simulink library "ammclib_bam_S32K3xx"  (R2016a)
(part 5 of 50)

      |     u16NShift_Q=15;
      |     warning(['Parameter u16NShift_Q of ' gcb ' exceeds the fixed-point range.']);
      |   end
      |   f16CC1sc_D=round(cc1fd*2^(-u16NShift_D)*2^15);
      |   if f16CC1sc_D>2^15-1
      |     f16CC1sc_D=2^15-1;
      |     warning(['Parameter f16CC1sc_D of ' gcb ' exceeds the fixed-point range.']);
      |   end
      |   if f16CC1sc_D<-2^15
      |     f16CC1sc_D=-2^15;
      |     warning(['Parameter f16CC1sc_D of ' gcb ' exceeds the fixed-point range.']);
      |   end
      |   f16CC2sc_D=round(cc2fd*2^(-u16NShift_D)*2^15);
      |   if f16CC2sc_D>2^15-1
      |     f16CC2sc_D=2^15-1;
      |     warning(['Parameter f16CC2sc_D of ' gcb ' exceeds the fixed-point range.']);
      |   end
      |   if f16CC2sc_D<-2^15
      |     f16CC2sc_D=-2^15;
      |     warning(['Parameter f16CC2sc_D of ' gcb ' exceeds the fixed-point range.']);
      |   end
      |   f16CC1sc_Q=round(cc1fq*2^(-u16NShift_Q)*2^15);
      |   if f16CC1sc_Q>2^15-1
      |     f16CC1sc_Q=2^15-1;
      |     warning(['Parameter f16CC1sc_Q of ' gcb ' exceeds the fixed-point range.']);
      |   end
      |   if f16CC1sc_Q<-2^15
      |     f16CC1sc_Q=-2^15;
      |     warning(['Parameter f16CC1sc_Q of ' gcb ' exceeds the fixed-point range.']);
      |   end
      |   f16CC2sc_Q=round(cc2fq*2^(-u16NShift_Q)*2^15);
      |   if f16CC2sc_Q>2^15-1
      |     f16CC2sc_Q=2^15-1;
      |     warning(['Parameter f16CC2sc_Q of ' gcb ' exceeds the fixed-point range.']);
      |   end
      |   if f16CC2sc_Q<-2^15
      |     f16CC2sc_Q=-2^15;
      |     warning(['Parameter f16CC2sc_Q of ' gcb ' exceeds the fixed-point range.']);
      |   end
      |   if isnan(f16CC1sc_D)
      |     if ~strcmp(f16CC1sc_D_bkup,'0')
      |       set_param(gcb,'f16CC1sc_D','0');
      |     end
      |   else
      |     tmps=num2str(f16CC1sc_D);
      |     if ~strcmp(f16CC1sc_D_bkup,tmps)
      |       set_param(gcb,'f16CC1sc_D',tmps);
      |     end
      |   end
      |   if isnan(f16CC2sc_D)
      |     if ~strcmp(f16CC2sc_D_bkup,'0')
      |       set_param(gcb,'f16CC2sc_D','0');
      |     end
      |   else
      |     tmps=num2str(f16CC2sc_D);
      |     if ~strcmp(f16CC2sc_D_bkup,tmps)
      |       set_param(gcb,'f16CC2sc_D',tmps);
      |     end
      |   end
      |   if isnan(u16NShift_D)
      |     if ~strcmp(u16NShift_D_bkup,'0')
      |       set_param(gcb,'u16NShift_D','0');
      |     end
      |   else
      |     tmps=num2str(u16NShift_D);
      |     if ~strcmp(u16NShift_D_bkup,tmps)
      |       set_param(gcb,'u16NShift_D',tmps);
      |     end
      |   end
      |   if isnan(f16CC1sc_Q)
      |     if ~strcmp(f16CC1sc_Q_bkup,'0')
      |       set_param(gcb,'f16CC1sc_Q','0');
      |     end
      |   else
      |     tmps=num2str(f16CC1sc_Q);
      |     if ~strcmp(f16CC1sc_Q_bkup,tmps)
      |       set_param(gcb,'f16CC1sc_Q',tmps);
      |     end
      |   end
      |   if isnan(f16CC2sc_Q)
      |     if ~strcmp(f16CC2sc_Q_bkup,'0')
      |       set_param(gcb,'f16CC2sc_Q','0');
      |     end
      |   else
      |     tmps=num2str(f16CC2sc_Q);
      |     if ~strcmp(f16CC2sc_Q_bkup,tmps)
      |       set_param(gcb,'f16CC2sc_Q',tmps);
      |     end
      |   end
      |   if isnan(u16NShift_Q)
      |     if ~strcmp(u16NShift_Q_bkup,'0')
      |       set_param(gcb,'u16NShift_Q','0');
      |     end
      |   else
      |     tmps=num2str(u16NShift_Q);
      |     if ~strcmp(u16NShift_Q_bkup,tmps)
      |       set_param(gcb,'u16NShift_Q',tmps);
      |     end
      |   end
      | end
      mask Callback iscale:
      | autoCalcEn=get_param(gcb,'autoCalcEn');
      | if strcmp(autoCalcEn,'on')
      |   SampleTime=Simulink.data.evalinGlobal(bdroot,get_param(gcb,'SampleTime'));
      |   if (SampleTime==-1)
      |     SampleTime=str2double(get_param(gcb,'SampleTime_1'));
      |   end
      |   f16CC1sc_D_bkup=get_param(gcb,'f16CC1sc_D');
      |   f16CC2sc_D_bkup=get_param(gcb,'f16CC2sc_D');
      |   u16NShift_D_bkup=get_param(gcb,'u16NShift_D');
      |   f16CC1sc_Q_bkup=get_param(gcb,'f16CC1sc_Q');
      |   f16CC2sc_Q_bkup=get_param(gcb,'f16CC2sc_Q');
      |   u16NShift_Q_bkup=get_param(gcb,'u16NShift_Q');
      |   intmethod=get_param(gcb,'intmethod');
      |   if0=Simulink.data.evalinGlobal(bdroot,get_param(gcb,'if0'));
      |   iksi=Simulink.data.evalinGlobal(bdroot,get_param(gcb,'iksi'));
      |   Ld=Simulink.data.evalinGlobal(bdroot,get_param(gcb,'Ld'));
      |   Lq=Simulink.data.evalinGlobal(bdroot,get_param(gcb,'Lq'));
      |   Rs=Simulink.data.evalinGlobal(bdroot,get_param(gcb,'Rs'));
      |   uscale=Simulink.data.evalinGlobal(bdroot,get_param(gcb,'uscale'));
      |   iscale=Simulink.data.evalinGlobal(bdroot,get_param(gcb,'iscale'));
      |   if (if0<=0)
      |     warning('Natural frequency f0 must be positive.');
      |   end
      |   if (iksi<=0)
      |     warning('Current loop attenuation must be positive.');
      |   end
      |   if (iksi>1)
      |     warning('Current loop attenuation must not exceed 1.');
      |   end
      |   if (Ld<=0)
      |     warning('Inductance Ld must be positive.');
      |   end
      |   if (Lq<=0)
      |     warning('Inductance Lq must be positive.');
      |   end
      |   if (Rs<0)
      |     warning('Resistance Rs must be non-negative.');
      |   end
      |   if (uscale<=0)
      |     warning('U_max must be positive.');
      |   end
      |   if (iscale<=0)
      |     warning('I_max must be positive.');
      |   end
      |   w0=6.283185307179586*if0;
      |   pgainD=2.0*iksi*w0*Ld-Rs;
      |   igainD=w0*w0*Ld;
      |   pgainQ=2.0*iksi*w0*Lq-Rs;
      |   igainQ=w0*w0*Lq;
      |   if strcmp(intmethod,'Forward Rectangular')
      |     cc1d=pgainD;
      |     cc2d=-pgainD+igainD*SampleTime;
      |     cc1q=pgainQ;
      |     cc2q=-pgainQ+igainQ*SampleTime;
      |   else
      |     if strcmp(intmethod,'Backward Rectangular')
      |       cc1d=pgainD+igainD*SampleTime;
      |       cc2d=-pgainD;
      |       cc1q=pgainQ+igainQ*SampleTime;
      |       cc2q=-pgainQ;
      |     else
      |       cc1d=pgainD+igainD*SampleTime*0.5;
      |       cc2d=-pgainD+igainD*SampleTime*0.5;
      |       cc1q=pgainQ+igainQ*SampleTime*0.5;
      |       cc2q=-pgainQ+igainQ*SampleTime*0.5;
      |     end
      |   end
      |   cc1fd=cc1d*iscale/uscale;
      |   cc2fd=cc2d*iscale/uscale;
      |   cc1fq=cc1q*iscale/uscale;
      |   cc2fq=cc2q*iscale/uscale;
      |   u16NShift_D=ceil(log2(abs(cc1fd)));
      |   tmpsh=ceil(log2(abs(cc2fd)));
      |   if u16NShift_D<tmpsh
      |     u16NShift_D=tmpsh;
      |   end
      |   if u16NShift_D<0
      |     u16NShift_D=0;
      |   end
      |   if u16NShift_D>15
      |     u16NShift_D=15;
      |     warning(['Parameter u16NShift_D of ' gcb ' exceeds the fixed-point range.']);
      |   end
      |   u16NShift_Q=ceil(log2(abs(cc1fq)));
      |   tmpsh=ceil(log2(abs(cc2fq)));
      |   if u16NShift_Q<tmpsh
      |     u16NShift_Q=tmpsh;
      |   end
      |   if u16NShift_Q<0
      |     u16NShift_Q=0;
      |   end
      |   if u16NShift_Q>15
      |     u16NShift_Q=15;
      |     warning(['Parameter u16NShift_Q of ' gcb ' exceeds the fixed-point range.']);
      |   end
      |   f16CC1sc_D=round(cc1fd*2^(-u16NShift_D)*2^15);
      |   if f16CC1sc_D>2^15-1
      |     f16CC1sc_D=2^15-1;
      |     warning(['Parameter f16CC1sc_D of ' gcb ' exceeds the fixed-point range.']);
      |   end
      |   if f16CC1sc_D<-2^15
      |     f16CC1sc_D=-2^15;
      |     warning(['Parameter f16CC1sc_D of ' gcb ' exceeds the fixed-point range.']);
      |   end
      |   f16CC2sc_D=round(cc2fd*2^(-u16NShift_D)*2^15);
      |   if f16CC2sc_D>2^15-1
      |     f16CC2sc_D=2^15-1;
      |     warning(['Parameter f16CC2sc_D of ' gcb ' exceeds the fixed-point range.']);
      |   end
      |   if f16CC2sc_D<-2^15
      |     f16CC2sc_D=-2^15;
      |     warning(['Parameter f16CC2sc_D of ' gcb ' exceeds the fixed-point range.']);
      |   end
      |   f16CC1sc_Q=round(cc1fq*2^(-u16NShift_Q)*2^15);
      |   if f16CC1sc_Q>2^15-1
      |     f16CC1sc_Q=2^15-1;
      |     warning(['Parameter f16CC1sc_Q of ' gcb ' exceeds the fixed-point range.']);
      |   end
      |   if f16CC1sc_Q<-2^15
      |     f16CC1sc_Q=-2^15;
      |     warning(['Parameter f16CC1sc_Q of ' gcb ' exceeds the fixed-point range.']);
      |   end
      |   f16CC2sc_Q=round(cc2fq*2^(-u16NShift_Q)*2^15);
      |   if f16CC2sc_Q>2^15-1
      |     f16CC2sc_Q=2^15-1;
      |     warning(['Parameter f16CC2sc_Q of ' gcb ' exceeds the fixed-point range.']);
      |   end
      |   if f16CC2sc_Q<-2^15
      |     f16CC2sc_Q=-2^15;
      |     warning(['Parameter f16CC2sc_Q of ' gcb ' exceeds the fixed-point range.']);
      |   end
      |   if isnan(f16CC1sc_D)
      |     if ~strcmp(f16CC1sc_D_bkup,'0')
      |       set_param(gcb,'f16CC1sc_D','0');
      |     end
      |   else
      |     tmps=num2str(f16CC1sc_D);
      |     if ~strcmp(f16CC1sc_D_bkup,tmps)
      |       set_param(gcb,'f16CC1sc_D',tmps);
      |     end
      |   end
      |   if isnan(f16CC2sc_D)
      |     if ~strcmp(f16CC2sc_D_bkup,'0')
      |       set_param(gcb,'f16CC2sc_D','0');
      |     end
      |   else
      |     tmps=num2str(f16CC2sc_D);
      |     if ~strcmp(f16CC2sc_D_bkup,tmps)
      |       set_param(gcb,'f16CC2sc_D',tmps);
      |     end
      |   end
      |   if isnan(u16NShift_D)
      |     if ~strcmp(u16NShift_D_bkup,'0')
      |       set_param(gcb,'u16NShift_D','0');
      |     end
      |   else
      |     tmps=num2str(u16NShift_D);
      |     if ~strcmp(u16NShift_D_bkup,tmps)
      |       set_param(gcb,'u16NShift_D',tmps);
      |     end
      |   end
      |   if isnan(f16CC1sc_Q)
      |     if ~strcmp(f16CC1sc_Q_bkup,'0')
      |       set_param(gcb,'f16CC1sc_Q','0');
      |     end
      |   else
      |     tmps=num2str(f16CC1sc_Q);
      |     if ~strcmp(f16CC1sc_Q_bkup,tmps)
      |       set_param(gcb,'f16CC1sc_Q',tmps);
      |     end
      |   end
      |   if isnan(f16CC2sc_Q)
      |     if ~strcmp(f16CC2sc_Q_bkup,'0')
      |       set_param(gcb,'f16CC2sc_Q','0');
      |     end
      |   else
      |     tmps=num2str(f16CC2sc_Q);
      |     if ~strcmp(f16CC2sc_Q_bkup,tmps)
      |       set_param(gcb,'f16CC2sc_Q',tmps);
      |     end
      |   end
      |   if isnan(u16NShift_Q)
      |     if ~strcmp(u16NShift_Q_bkup,'0')
      |       set_param(gcb,'u16NShift_Q','0');
      |     end
      |   else
      |     tmps=num2str(u16NShift_Q);
      |     if ~strcmp(u16NShift_Q_bkup,tmps)
      |       set_param(gcb,'u16NShift_Q',tmps);
      |     end
      |   end
      | end
      mask Callback autoCalcEn:
      | maskStr=get_param(gcb,'showStates');
      | if strcmp(maskStr,'Hide (faster execution)')
      |   p=Simulink.Mask.get(gcb);
      |   autoCalcEn=get_param(gcb,'autoCalcEn');
      |   hintText=p.getDialogControl('timeHint');
      |   if strcmp(autoCalcEn,'on')
      |     param=p.getParameter('iscale');
      |     if strcmp(param.Enabled,'off')
      |       SampleTime=Simulink.data.evalinGlobal(bdroot,get_param(gcb,'SampleTime'));
      |       if SampleTime==-1
      |         SampleTime=str2double(get_param(gcb,'SampleTime_1'));
      |         if isnan(SampleTime)
      |           hintText.Prompt=['Note: Implementation parameters cannot be calculated yet because the block''s inherited sample time is unknown. Simulink will update the sample time when you run the simulation.'];
      |         else
      |           hintText.Prompt=['Caution: Implementation parameters depend on inherited sample time. Make sure that the sample time of the block''s inputs corresponds to the sampling period in the target application.'];
      |         end
      |       else
      |         hintText.Prompt='Caution: Implementation parameters depend on the sample time. Make sure that the simulation time step corresponds to the sampling period in the target application.';
      |       end
      |       p=Simulink.Mask.get(gcb);
      |       param=p.getParameter('intmethod');
      |       param.set('Enabled','on');
      |       param=p.getParameter('if0');
      |       param.set('Enabled','on');
      |       param=p.getParameter('iksi');
      |       param.set('Enabled','on');
      |       param=p.getParameter('Ld');
      |       param.set('Enabled','on');
      |       param=p.getParameter('Lq');
      |       param.set('Enabled','on');
      |       param=p.getParameter('Rs');
      |       param.set('Enabled','on');
      |       param=p.getParameter('uscale');
      |       param.set('Enabled','on');
      |       param=p.getParameter('iscale');
      |       param.set('Enabled','on');
      |     else
      |       SampleTime=Simulink.data.evalinGlobal(bdroot,get_param(gcb,'SampleTime'));
      |       if SampleTime==-1
      |         SampleTime=str2double(get_param(gcb,'SampleTime_1'));
      |       end
      |     end
      |     f16CC1sc_D_bkup=get_param(gcb,'f16CC1sc_D');
      |     f16CC2sc_D_bkup=get_param(gcb,'f16CC2sc_D');
      |     u16NShift_D_bkup=get_param(gcb,'u16NShift_D');
      |     f16CC1sc_Q_bkup=get_param(gcb,'f16CC1sc_Q');
      |     f16CC2sc_Q_bkup=get_param(gcb,'f16CC2sc_Q');
      |     u16NShift_Q_bkup=get_param(gcb,'u16NShift_Q');
      |     intmethod=get_param(gcb,'intmethod');
      |     if0=Simulink.data.evalinGlobal(bdroot,get_param(gcb,'if0'));
      |     iksi=Simulink.data.evalinGlobal(bdroot,get_param(gcb,'iksi'));
      |     Ld=Simulink.data.evalinGlobal(bdroot,get_param(gcb,'Ld'));
      |     Lq=Simulink.data.evalinGlobal(bdroot,get_param(gcb,'Lq'));
      |     Rs=Simulink.data.evalinGlobal(bdroot,get_param(gcb,'Rs'));
      |     uscale=Simulink.data.evalinGlobal(bdroot,get_param(gcb,'uscale'));
      |     iscale=Simulink.data.evalinGlobal(bdroot,get_param(gcb,'iscale'));
      |     if (if0<=0)
      |       warning('Natural frequency f0 must be positive.');
      |     end
      |     if (iksi<=0)
      |       warning('Current loop attenuation must be positive.');
      |     end
      |     if (iksi>1)
      |       warning('Current loop attenuation must not exceed 1.');
      |     end
      |     if (Ld<=0)
      |       warning('Inductance Ld must be positive.');
      |     end
      |     if (Lq<=0)
      |       warning('Inductance Lq must be positive.');
      |     end
      |     if (Rs<0)
      |       warning('Resistance Rs must be non-negative.');
      |     end
      |     if (uscale<=0)
      |       warning('U_max must be positive.');
      |     end
      |     if (iscale<=0)
      |       warning('I_max must be positive.');
      |     end
      |     w0=6.283185307179586*if0;
      |     pgainD=2.0*iksi*w0*Ld-Rs;
      |     igainD=w0*w0*Ld;
      |     pgainQ=2.0*iksi*w0*Lq-Rs;
      |     igainQ=w0*w0*Lq;
      |     if strcmp(intmethod,'Forward Rectangular')
      |       cc1d=pgainD;
      |       cc2d=-pgainD+igainD*SampleTime;
      |       cc1q=pgainQ;
      |       cc2q=-pgainQ+igainQ*SampleTime;
      |     else
      |       if strcmp(intmethod,'Backward Rectangular')
      |         cc1d=pgainD+igainD*SampleTime;
      |         cc2d=-pgainD;
      |         cc1q=pgainQ+igainQ*SampleTime;
      |         cc2q=-pgainQ;
      |       else
      |         cc1d=pgainD+igainD*SampleTime*0.5;
      |         cc2d=-pgainD+igainD*SampleTime*0.5;
      |         cc1q=pgainQ+igainQ*SampleTime*0.5;
      |         cc2q=-pgainQ+igainQ*SampleTime*0.5;
      |       end
      |     end
      |     cc1fd=cc1d*iscale/uscale;
      |     cc2fd=cc2d*iscale/uscale;
      |     cc1fq=cc1q*iscale/uscale;
      |     cc2fq=cc2q*iscale/uscale;
      |     u16NShift_D=ceil(log2(abs(cc1fd)));
      |     tmpsh=ceil(log2(abs(cc2fd)));
      |     if u16NShift_D<tmpsh
      |       u16NShift_D=tmpsh;
      |     end
      |     if u16NShift_D<0
      |       u16NShift_D=0;
      |     end
      |     if u16NShift_D>15
      |       u16NShift_D=15;
      |       warning(['Parameter u16NShift_D of ' gcb ' exceeds the fixed-point range.']);
      |     end
      |     u16NShift_Q=ceil(log2(abs(cc1fq)));
      |     tmpsh=ceil(log2(abs(cc2fq)));
      |     if u16NShift_Q<tmpsh
      |       u16NShift_Q=tmpsh;
      |     end
      |     if u16NShift_Q<0
      |       u16NShift_Q=0;
      |     end
      |     if u16NShift_Q>15
      |       u16NShift_Q=15;
      |       warning(['Parameter u16NShift_Q of ' gcb ' exceeds the fixed-point range.']);
      |     end
      |     f16CC1sc_D=round(cc1fd*2^(-u16NShift_D)*2^15);
      |     if f16CC1sc_D>2^15-1
      |       f16CC1sc_D=2^15-1;
      |       warning(['Parameter f16CC1sc_D of ' gcb ' exceeds the fixed-point range.']);
      |     end
      |     if f16CC1sc_D<-2^15
      |       f16CC1sc_D=-2^15;
      |       warning(['Parameter f16CC1sc_D of ' gcb ' exceeds the fixed-point range.']);
      |     end
      |     f16CC2sc_D=round(cc2fd*2^(-u16NShift_D)*2^15);
      |     if f16CC2sc_D>2^15-1
      |       f16CC2sc_D=2^15-1;
      |       warning(['Parameter f16CC2sc_D of ' gcb ' exceeds the fixed-point range.']);
      |     end
      |     if f16CC2sc_D<-2^15
      |       f16CC2sc_D=-2^15;
      |       warning(['Parameter f16CC2sc_D of ' gcb ' exceeds the fixed-point range.']);
      |     end
      |     f16CC1sc_Q=round(cc1fq*2^(-u16NShift_Q)*2^15);
      |     if f16CC1sc_Q>2^15-1
      |       f16CC1sc_Q=2^15-1;
      |       warning(['Parameter f16CC1sc_Q of ' gcb ' exceeds the fixed-point range.']);
      |     end
      |     if f16CC1sc_Q<-2^15
      |       f16CC1sc_Q=-2^15;
      |       warning(['Parameter f16CC1sc_Q of ' gcb ' exceeds the fixed-point range.']);
      |     end
      |     f16CC2sc_Q=round(cc2fq*2^(-u16NShift_Q)*2^15);
      |     if f16CC2sc_Q>2^15-1
      |       f16CC2sc_Q=2^15-1;
      |       warning(['Parameter f16CC2sc_Q of ' gcb ' exceeds the fixed-point range.']);
      |     end
      |     if f16CC2sc_Q<-2^15
      |       f16CC2sc_Q=-2^15;
      |       warning(['Parameter f16CC2sc_Q of ' gcb ' exceeds the fixed-point range.']);
      |     end
      |     if isnan(f16CC1sc_D)
      |       if ~strcmp(f16CC1sc_D_bkup,'0')
      |         set_param(gcb,'f16CC1sc_D','0');
      |       end
      |     else
      |       tmps=num2str(f16CC1sc_D);
      |       if ~strcmp(f16CC1sc_D_bkup,tmps)
      |         set_param(gcb,'f16CC1sc_D',tmps);
      |       end
      |     end
      |     if isnan(f16CC2sc_D)
      |       if ~strcmp(f16CC2sc_D_bkup,'0')
      |         set_param(gcb,'f16CC2sc_D','0');
      |       end
      |     else
      |       tmps=num2str(f16CC2sc_D);
      |       if ~strcmp(f16CC2sc_D_bkup,tmps)
      |         set_param(gcb,'f16CC2sc_D',tmps);
      |       end
      |     end
      |     if isnan(u16NShift_D)
      |       if ~strcmp(u16NShift_D_bkup,'0')
      |         set_param(gcb,'u16NShift_D','0');
      |       end
      |     else
      |       tmps=num2str(u16NShift_D);
      |       if ~strcmp(u16NShift_D_bkup,tmps)
      |         set_param(gcb,'u16NShift_D',tmps);
      |       end
      |     end
      |     if isnan(f16CC1sc_Q)
      |       if ~strcmp(f16CC1sc_Q_bkup,'0')
      |         set_param(gcb,'f16CC1sc_Q','0');
      |       end
      |     else
      |       tmps=num2str(f16CC1sc_Q);
      |       if ~strcmp(f16CC1sc_Q_bkup,tmps)
      |         set_param(gcb,'f16CC1sc_Q',tmps);
      |       end
      |     end
      |     if isnan(f16CC2sc_Q)
      |       if ~strcmp(f16CC2sc_Q_bkup,'0')
      |         set_param(gcb,'f16CC2sc_Q','0');
      |       end
      |     else
      |       tmps=num2str(f16CC2sc_Q);
      |       if ~strcmp(f16CC2sc_Q_bkup,tmps)
      |         set_param(gcb,'f16CC2sc_Q',tmps);
      |       end
      |     end
      |     if isnan(u16NShift_Q)
      |       if ~strcmp(u16NShift_Q_bkup,'0')
      |         set_param(gcb,'u16NShift_Q','0');
      |       end
      |     else
      |       tmps=num2str(u16NShift_Q);
      |       if ~strcmp(u16NShift_Q_bkup,tmps)
      |         set_param(gcb,'u16NShift_Q',tmps);
      |       end
      |     end
      |   else
      |     param=p.getParameter('iscale');
      |     if strcmp(param.Enabled,'on')
      |       hintText.Prompt='Caution: Implementation parameters are fixed.';
      |       p=Simulink.Mask.get(gcb);
      |       param=p.getParameter('intmethod');
      |       param.set('Enabled','off');
      |       param=p.getParameter('if0');
      |       param.set('Enabled','off');
      |       param=p.getParameter('iksi');
      |       param.set('Enabled','off');
      |       param=p.getParameter('Ld');
      |       param.set('Enabled','off');
      |       param=p.getParameter('Lq');
      |       param.set('Enabled','off');
      |       param=p.getParameter('Rs');
      |       param.set('Enabled','off');
      |       param=p.getParameter('uscale');
      |       param.set('Enabled','off');
      |       param=p.getParameter('iscale');
      |       param.set('Enabled','off');
      |     end
      |   end
      | end
      mask DialogControl CompBut Prompt: Recalculate sample times
      mask DialogControl CompBut Tooltip: Simulink updates the sample times of all blocks when the simulation is run. This button will update the sample times now.
      mask DialogControl CompBut Callback:
      | btn=questdlg('This will apply all changes in all open dialog boxes and update the schematic. Do you want to proceed?','Apply all changes','Continue','Cancel','Continue');
      | if strcmp(btn,'Continue')
      |   dlgs=DAStudio.ToolRoot.getOpenDialogs;
      |   for i=1:length(dlgs)
      |     dlgs(i).apply;
      |   end
      |   try
      |     SampleTime_1=str2double(get_param(gcb,'SampleTime_1'));
      |     ts=Simulink.Block.getSampleTimes(gcb);
      |     ts=ts(1).Value(1);
      |     if (SampleTime_1 ~= ts)
      |       SampleTime_1=ts;
      |       set_param(gcb,'SampleTime_1',num2str(ts));
      |       autoCalcEn=get_param(gcb,'autoCalcEn');
      |       if strcmp(autoCalcEn,'on')
      |         SampleTime=Simulink.data.evalinGlobal(bdroot,get_param(gcb,'SampleTime'));
      |         p=Simulink.Mask.get(gcb);
      |         hintText=p.getDialogControl('timeHint');
      |         if SampleTime==-1
      |           SampleTime=SampleTime_1;
      |           hintText.Prompt='Caution: Implementation parameters depend on inherited sample time. Make sure that the sample time of the block''s inputs corresponds to the sampling period in the target application.';
      |         else
      |           hintText.Prompt='Caution: Implementation parameters depend on the sample time. Make sure that the simulation time step corresponds to the sampling period in the target application.';
      |         end
      |         f16CC1sc_D_bkup=get_param(gcb,'f16CC1sc_D');
      |         f16CC2sc_D_bkup=get_param(gcb,'f16CC2sc_D');
      |         u16NShift_D_bkup=get_param(gcb,'u16NShift_D');
      |         f16CC1sc_Q_bkup=get_param(gcb,'f16CC1sc_Q');
      |         f16CC2sc_Q_bkup=get_param(gcb,'f16CC2sc_Q');
      |         u16NShift_Q_bkup=get_param(gcb,'u16NShift_Q');
      |         intmethod=get_param(gcb,'intmethod');
      |         if0=Simulink.data.evalinGlobal(bdroot,get_param(gcb,'if0'));
      |         iksi=Simulink.data.evalinGlobal(bdroot,get_param(gcb,'iksi'));
      |         Ld=Simulink.data.evalinGlobal(bdroot,get_param(gcb,'Ld'));
      |         Lq=Simulink.data.evalinGlobal(bdroot,get_param(gcb,'Lq'));
      |         Rs=Simulink.data.evalinGlobal(bdroot,get_param(gcb,'Rs'));
      |         uscale=Simulink.data.evalinGlobal(bdroot,get_param(gcb,'uscale'));
      |         iscale=Simulink.data.evalinGlobal(bdroot,get_param(gcb,'iscale'));
      |         if (if0<=0)
      |           warning('Natural frequency f0 must be positive.');
      |         end
      |         if (iksi<=0)
      |           warning('Current loop attenuation must be positive.');
      |         end
      |         if (iksi>1)
      |           warning('Current loop attenuation must not exceed 1.');
      |         end
      |         if (Ld<=0)
      |           warning('Inductance Ld must be positive.');
      |         end
      |         if (Lq<=0)
      |           warning('Inductance Lq must be positive.');
      |         end
      |         if (Rs<0)
      |           warning('Resistance Rs must be non-negative.');
      |         end
      |         if (uscale<=0)
      |           warning('U_max must be positive.');
      |         end
      |         if (iscale<=0)
      |           warning('I_max must be positive.');
      |         end
      |         w0=6.283185307179586*if0;
      |         pgainD=2.0*iksi*w0*Ld-Rs;
      |         igainD=w0*w0*Ld;
      |         pgainQ=2.0*iksi*w0*Lq-Rs;
      |         igainQ=w0*w0*Lq;
      |         if strcmp(intmethod,'Forward Rectangular')
      |           cc1d=pgainD;
      |           cc2d=-pgainD+igainD*SampleTime;
      |           cc1q=pgainQ;
      |           cc2q=-pgainQ+igainQ*SampleTime;
      |         else
      |           if strcmp(intmethod,'Backward Rectangular')
      |             cc1d=pgainD+igainD*SampleTime;
      |             cc2d=-pgainD;
      |             cc1q=pgainQ+igainQ*SampleTime;
      |             cc2q=-pgainQ;
      |           else
      |             cc1d=pgainD+igainD*SampleTime*0.5;
      |             cc2d=-pgainD+igainD*SampleTime*0.5;
      |             cc1q=pgainQ+igainQ*SampleTime*0.5;
      |             cc2q=-pgainQ+igainQ*SampleTime*0.5;
      |           end
      |         end
      |         cc1fd=cc1d*iscale/uscale;
      |         cc2fd=cc2d*iscale/uscale;
      |         cc1fq=cc1q*iscale/uscale;
      |         cc2fq=cc2q*iscale/uscale;
      |         u16NShift_D=ceil(log2(abs(cc1fd)));
      |         tmpsh=ceil(log2(abs(cc2fd)));
      |         if u16NShift_D<tmpsh
      |           u16NShift_D=tmpsh;
      |         end
      |         if u16NShift_D<0
      |           u16NShift_D=0;
      |         end
      |         if u16NShift_D>15
      |           u16NShift_D=15;
      |           warning(['Parameter u16NShift_D of ' gcb ' exceeds the fixed-point range.']);
      |         end
      |         u16NShift_Q=ceil(log2(abs(cc1fq)));
      |         tmpsh=ceil(log2(abs(cc2fq)));
      |         if u16NShift_Q<tmpsh
      |           u16NShift_Q=tmpsh;
      |         end
      |         if u16NShift_Q<0
      |           u16NShift_Q=0;
      |         end
      |         if u16NShift_Q>15
      |           u16NShift_Q=15;
      |           warning(['Parameter u16NShift_Q of ' gcb ' exceeds the fixed-point range.']);
      |         end
      |         f16CC1sc_D=round(cc1fd*2^(-u16NShift_D)*2^15);
      |         if f16CC1sc_D>2^15-1
      |           f16CC1sc_D=2^15-1;
      |           warning(['Parameter f16CC1sc_D of ' gcb ' exceeds the fixed-point range.']);
      |         end
      |         if f16CC1sc_D<-2^15
      |           f16CC1sc_D=-2^15;
      |           warning(['Parameter f16CC1sc_D of ' gcb ' exceeds the fixed-point range.']);
      |         end
      |         f16CC2sc_D=round(cc2fd*2^(-u16NShift_D)*2^15);
      |         if f16CC2sc_D>2^15-1
      |           f16CC2sc_D=2^15-1;
      |           warning(['Parameter f16CC2sc_D of ' gcb ' exceeds the fixed-point range.']);
      |         end
      |         if f16CC2sc_D<-2^15
      |           f16CC2sc_D=-2^15;
      |           warning(['Parameter f16CC2sc_D of ' gcb ' exceeds the fixed-point range.']);
      |         end
      |         f16CC1sc_Q=round(cc1fq*2^(-u16NShift_Q)*2^15);
      |         if f16CC1sc_Q>2^15-1
      |           f16CC1sc_Q=2^15-1;
      |           warning(['Parameter f16CC1sc_Q of ' gcb ' exceeds the fixed-point range.']);
      |         end
      |         if f16CC1sc_Q<-2^15
      |           f16CC1sc_Q=-2^15;
      |           warning(['Parameter f16CC1sc_Q of ' gcb ' exceeds the fixed-point range.']);
      |         end
      |         f16CC2sc_Q=round(cc2fq*2^(-u16NShift_Q)*2^15);
      |         if f16CC2sc_Q>2^15-1
      |           f16CC2sc_Q=2^15-1;
      |           warning(['Parameter f16CC2sc_Q of ' gcb ' exceeds the fixed-point range.']);
      |         end
      |         if f16CC2sc_Q<-2^15
      |           f16CC2sc_Q=-2^15;
      |           warning(['Parameter f16CC2sc_Q of ' gcb ' exceeds the fixed-point range.']);
      |         end
      |         if isnan(f16CC1sc_D)
      |           if ~strcmp(f16CC1sc_D_bkup,'0')
      |             set_param(gcb,'f16CC1sc_D','0');
      |           end
      |         else
      |           tmps=num2str(f16CC1sc_D);
      |           if ~strcmp(f16CC1sc_D_bkup,tmps)
      |             set_param(gcb,'f16CC1sc_D',tmps);
      |           end
      |         end
      |         if isnan(f16CC2sc_D)
      |           if ~strcmp(f16CC2sc_D_bkup,'0')
      |             set_param(gcb,'f16CC2sc_D','0');
      |           end
      |         else
      |           tmps=num2str(f16CC2sc_D);
      |           if ~strcmp(f16CC2sc_D_bkup,tmps)
      |             set_param(gcb,'f16CC2sc_D',tmps);
      |           end
      |         end
      |         if isnan(u16NShift_D)
      |           if ~strcmp(u16NShift_D_bkup,'0')
      |             set_param(gcb,'u16NShift_D','0');
      |           end
      |         else
      |           tmps=num2str(u16NShift_D);
      |           if ~strcmp(u16NShift_D_bkup,tmps)
      |             set_param(gcb,'u16NShift_D',tmps);
      |           end
      |         end
      |         if isnan(f16CC1sc_Q)
      |           if ~strcmp(f16CC1sc_Q_bkup,'0')
      |             set_param(gcb,'f16CC1sc_Q','0');
      |           end
      |         else
      |           tmps=num2str(f16CC1sc_Q);
      |           if ~strcmp(f16CC1sc_Q_bkup,tmps)
      |             set_param(gcb,'f16CC1sc_Q',tmps);
      |           end
      |         end
      |         if isnan(f16CC2sc_Q)
      |           if ~strcmp(f16CC2sc_Q_bkup,'0')
      |             set_param(gcb,'f16CC2sc_Q','0');
      |           end
      |         else
      |           tmps=num2str(f16CC2sc_Q);
      |           if ~strcmp(f16CC2sc_Q_bkup,tmps)
      |             set_param(gcb,'f16CC2sc_Q',tmps);
      |           end
      |         end
      |         if isnan(u16NShift_Q)
      |           if ~strcmp(u16NShift_Q_bkup,'0')
      |             set_param(gcb,'u16NShift_Q','0');
      |           end
      |         else
      |           tmps=num2str(u16NShift_Q);
      |           if ~strcmp(u16NShift_Q_bkup,tmps)
      |             set_param(gcb,'u16NShift_Q',tmps);
      |           end
      |         end
      |       end
      |     end
      |   catch
      |    warning(['Sample time cannot be calculated for the block ' gcb])
      |   end
      | end
      mask DialogControl timeHint Prompt: Note: Implementation parameters cannot be calculated yet because the block's inherited sample time is unknown. Simulink will update the sample time when you run the simulation.
      mask Display:
      | color('black');
      | pos = get_param(gcb, 'Position');
      | width = pos(3) - pos(1);
      | height = pos(4) - pos(2);
      | tX=width/2;
      | tY=height - 25;
      | color('black');
      | text(tX,tY, 'AMCLIB_CurrentLoop_F16', 'horizontalAlignment', 'center');
      | if showStates == 2
      |   color('red');
      |   text(tX,tY - 20, ['debugging mode' char(13) char(10) '(limited performance)'], 'horizontalAlignment', 'center');
      | end
  AMCLIB_FWSpeedLoop_F16 : Subsystem  StartFcn=|  TreatAsAtomicUnit=on  mask(AMCLIB_FWSpeedLoop_F16){showStates=Hide (faster execution), resetStatesEnable=Pre-set according to the first set of inputs after reset, showDebugOutputs=Hide, f32State_Out_showOutput=off, SampleTime=-1, wf0=30, wksi=1, J=1.6e-5, Kt=0.067, lambdaW=0.9, lambdaFW=0.9, Idmax=-5, ramprpm=6, mechspeed=3000, polepairs=1, uscale=15, iscale=10, autoCalcEn=on, u16NSamplesW=0, u16NSamplesFW=0, f16PropGainQ=0, f16IntegGainQ=0, s16PropGainShiftQ=0, s16IntegGainShiftQ=0, f16LowerLimitQ=0, f16UpperLimitQ=0, f16PropGainFW=0, f16IntegGainFW=0, s16PropGainShiftFW=0, s16IntegGainShiftFW=0, f16LowerLimitFW=0, f16UpperLimitFW=0, f32RampUp=0, f32RampDown=0, SampleTime_1=NaN}
      | ts=get_param(gcb,'CompiledSampleTime');
      | if iscell(ts)
      |   ts=ts{1};
      |   if iscell(ts)
      |     ts=ts{1};
      |   end
      | end
      | ts=ts(1);
      | set_param(gcb,'SampleTime_1',num2str(ts));
      | p=Simulink.Mask.get(gcb);
      | hintText=p.getDialogControl('timeHint');
      | SampleTime=Simulink.data.evalinGlobal(bdroot,get_param(gcb,'SampleTime'));
      | p=Simulink.Mask.get(gcb);
      | autoCalcEn=get_param(gcb,'autoCalcEn');
      | if strcmp(autoCalcEn,'on')
      |   if SampleTime==-1
      |     hintText.Prompt='Caution: Implementation parameters depend on inherited sample time. Make sure that the sample time of the block''s inputs corresponds to the sampling period in the target application.';
      |   else
      |     hintText.Prompt='Caution: Implementation parameters depend on the sample time. Make sure that the simulation time step corresponds to the sampling period in the target application.';
      |   end
      |   SampleTime=ts;
      |   u16NSamplesW_bkup=get_param(gcb,'u16NSamplesW');
      |   u16NSamplesFW_bkup=get_param(gcb,'u16NSamplesFW');
      |   f16PropGainQ_bkup=get_param(gcb,'f16PropGainQ');
      |   f16IntegGainQ_bkup=get_param(gcb,'f16IntegGainQ');
      |   s16PropGainShiftQ_bkup=get_param(gcb,'s16PropGainShiftQ');
      |   s16IntegGainShiftQ_bkup=get_param(gcb,'s16IntegGainShiftQ');
      |   f16LowerLimitQ_bkup=get_param(gcb,'f16LowerLimitQ');
      |   f16UpperLimitQ_bkup=get_param(gcb,'f16UpperLimitQ');
      |   f16PropGainFW_bkup=get_param(gcb,'f16PropGainFW');
      |   f16IntegGainFW_bkup=get_param(gcb,'f16IntegGainFW');
      |   s16PropGainShiftFW_bkup=get_param(gcb,'s16PropGainShiftFW');
      |   s16IntegGainShiftFW_bkup=get_param(gcb,'s16IntegGainShiftFW');
      |   f16LowerLimitFW_bkup=get_param(gcb,'f16LowerLimitFW');
      |   f16UpperLimitFW_bkup=get_param(gcb,'f16UpperLimitFW');
      |   f32RampUp_bkup=get_param(gcb,'f32RampUp');
      |   f32RampDown_bkup=get_param(gcb,'f32RampDown');
      |   wf0=Simulink.data.evalinGlobal(bdroot,get_param(gcb,'wf0'));
      |   wksi=Simulink.data.evalinGlobal(bdroot,get_param(gcb,'wksi'));
      |   J=Simulink.data.evalinGlobal(bdroot,get_param(gcb,'J'));
      |   Kt=Simulink.data.evalinGlobal(bdroot,get_param(gcb,'Kt'));
      |   lambdaW=Simulink.data.evalinGlobal(bdroot,get_param(gcb,'lambdaW'));
      |   lambdaFW=Simulink.data.evalinGlobal(bdroot,get_param(gcb,'lambdaFW'));
      |   Idmax=Simulink.data.evalinGlobal(bdroot,get_param(gcb,'Idmax'));
      |   ramprpm=Simulink.data.evalinGlobal(bdroot,get_param(gcb,'ramprpm'));
      |   mechspeed=Simulink.data.evalinGlobal(bdroot,get_param(gcb,'mechspeed'));
      |   polepairs=Simulink.data.evalinGlobal(bdroot,get_param(gcb,'polepairs'));
      |   uscale=Simulink.data.evalinGlobal(bdroot,get_param(gcb,'uscale'));
      |   iscale=Simulink.data.evalinGlobal(bdroot,get_param(gcb,'iscale'));
      |   if (wf0<=0)
      |     warning('Natural frequency f0 must be positive.');
      |   end
      |   if (wksi<=0)
      |     warning('Current loop attenuation must be positive.');
      |   end
      |   if (wksi>1)
      |     warning('Current loop attenuation must not exceed 1.');
      |   end
      |   if (J<=0)
      |     warning('Moment of inertia J must be positive.');
      |   end
      |   if (Kt<=0)
      |     warning('Torque constant Kt must be positive.');
      |   end
      |   if (lambdaW<0)
      |     warning('MA filter smoothing factor must be in the range 0..1.');
      |   end
      |   if (lambdaW>1)
      |     warning('MA filter smoothing factor must be in the range 0..1.');
      |   end
      |   if (lambdaFW<0)
      |     warning('MA filter smoothing factor must be in the range 0..1.');
      |   end
      |   if (lambdaFW>1)
      |     warning('MA filter smoothing factor must be in the range 0..1.');
      |   end
      |   if (mechspeed<=0)
      |     warning('Max. speed must be positive.');
      |   end
      |   if (polepairs<1)
      |     warning('Number of pole pairs must be a natural number (1, 2, 3, ...).');
      |   end
      |   if (round(polepairs)~=polepairs)
      |     warning('Number of pole pairs must be a natural number (1, 2, 3, ...).');
      |   end
      |   if (uscale<=0)
      |     warning('U_max must be positive.');
      |   end
      |   if (iscale<=0)
      |     warning('I_max must be positive.');
      |   end
      |   w0=6.283185307179586*wf0;
      |   pgain=2.0*wksi*w0*J/Kt;
      |   igain=w0*w0*J/Kt;
      |   wmax=polepairs*mechspeed*0.1047197551196598;
      |   kpf=pgain*wmax/iscale;
      |   s16PropGainShiftQ=ceil(log2(abs(kpf)));
      |   if s16PropGainShiftQ<-15
      |     s16PropGainShiftQ=-15;
      |   end
      |   if s16PropGainShiftQ>15
      |     s16PropGainShiftQ=15;
      |     warning(['Parameter s16PropGainShiftQ of ' gcb ' exceeds the fixed-point range.']);
      |   end
      |   f16PropGainQ=round(kpf*2^(-s16PropGainShiftQ)*2^15);
      |   if f16PropGainQ>2^15-1
      |     f16PropGainQ=2^15-1;
      |     warning(['Parameter f16PropGainQ of ' gcb ' exceeds the fixed-point range.']);
      |   end
      |   if f16PropGainQ<-2^15
      |     f16PropGainQ=-2^15;
      |     warning(['Parameter f16PropGainQ of ' gcb ' exceeds the fixed-point range.']);
      |   end
      |   kif=igain*SampleTime*0.5*wmax/iscale;
      |   s16IntegGainShiftQ=ceil(log2(abs(kif)));
      |   if s16IntegGainShiftQ<-15
      |     s16IntegGainShiftQ=-15;
      |   end
      |   if s16IntegGainShiftQ>15
      |     s16IntegGainShiftQ=15;
      |     warning(['Parameter s16IntegGainShiftQ of ' gcb ' exceeds the fixed-point range.']);
      |   end
      |   f16IntegGainQ=round(kif*2^(-s16IntegGainShiftQ)*2^15);
      |   if f16IntegGainQ>2^15-1
      |     f16IntegGainQ=2^15-1;
      |     warning(['Parameter f16IntegGainQ of ' gcb ' exceeds the fixed-point range.']);
      |   end
      |   if f16IntegGainQ<-2^15
      |     f16IntegGainQ=-2^15;
      |     warning(['Parameter f16IntegGainQ of ' gcb ' exceeds the fixed-point range.']);
      |   end
      |   f16LowerLimitQ=-32768;
      |   f16UpperLimitQ=32767;
      |   fwkpf=0.9*pgain*wmax/iscale;
      |   s16PropGainShiftFW=ceil(log2(abs(fwkpf)));
      |   if s16PropGainShiftFW<-15
      |     s16PropGainShiftFW=-15;
      |   end
      |   if s16PropGainShiftFW>15
      |     s16PropGainShiftFW=15;
      |     warning(['Parameter s16PropGainShiftFW of ' gcb ' exceeds the fixed-point range.']);
      |   end
      |   f16PropGainFW=round(fwkpf*2^(-s16PropGainShiftFW)*2^15);
      |   if f16PropGainFW>2^15-1
      |     f16PropGainFW=2^15-1;
      |     warning(['Parameter f16PropGainFW of ' gcb ' exceeds the fixed-point range.']);
      |   end
      |   if f16PropGainFW<-2^15
      |     f16PropGainFW=-2^15;
      |     warning(['Parameter f16PropGainFW of ' gcb ' exceeds the fixed-point range.']);
      |   end
      |   s16IntegGainShiftFW=s16IntegGainShiftQ;
      |   f16IntegGainFW=f16IntegGainQ;
      |   if (Idmax<0)
      |     iratio=abs(Idmax)/iscale;
      |     if (abs(iratio) > 1)
      |       iratio = 0;
      |     end
      |     lowlim=0.3183098861837907*acos(iratio)-0.5;
      |   else
      |     lowlim=0.0;
      |   end
      |   f16LowerLimitFW=round(lowlim*2^15);
      |   if f16LowerLimitFW>2^15-1
      |     f16LowerLimitFW=2^15-1;
      |     warning(['Parameter f16LowerLimitFW of ' gcb ' exceeds the fixed-point range.']);
      |   end
      |   if f16LowerLimitFW<-2^15
      |     f16LowerLimitFW=-2^15;
      |     warning(['Parameter f16LowerLimitFW of ' gcb ' exceeds the fixed-point range.']);
      |   end
      |   f16UpperLimitFW=0;
      |   u16NSamplesW=round(log2(1.0/abs(lambdaW)));
      |   if u16NSamplesW>15
      |     u16NSamplesW=15;
      |   end
      |   if u16NSamplesW<0
      |     u16NSamplesW=0;
      |   end
      |   u16NSamplesFW=round(log2(1.0/abs(lambdaFW)));
      |   if u16NSamplesFW>15
      |     u16NSamplesFW=15;
      |   end
      |   if u16NSamplesFW<0
      |     u16NSamplesFW=0;
      |   end
      |   rampsc=polepairs*abs(ramprpm)*0.1047197551196598/wmax;
      |   f32RampUp=round(rampsc*2^31);
      |   if f32RampUp>2^31-1
      |     f32RampUp=2^31-1;
      |     warning(['Parameter f32RampUp of ' gcb ' exceeds the fixed-point range.']);
      |   end
      |   if f32RampUp<-2^31
      |     f32RampUp=-2^31;
      |     warning(['Parameter f32RampUp of ' gcb ' exceeds the fixed-point range.']);
      |   end
      |   f32RampDown=round(rampsc*2^31);
      |   if f32RampDown>2^31-1
      |     f32RampDown=2^31-1;
      |     warning(['Parameter f32RampDown of ' gcb ' exceeds the fixed-point range.']);
      |   end
      |   if f32RampDown<-2^31
      |     f32RampDown=-2^31;
      |     warning(['Parameter f32RampDown of ' gcb ' exceeds the fixed-point range.']);
      |   end
      |   if isnan(u16NSamplesW)
      |     if ~strcmp(u16NSamplesW_bkup,'0')
      |       set_param(gcb,'u16NSamplesW','0');
      |     end
      |   else
      |     tmps=num2str(u16NSamplesW);
      |     if ~strcmp(u16NSamplesW_bkup,tmps)
      |       set_param(gcb,'u16NSamplesW',tmps);
      |     end
      |   end
      |   if isnan(u16NSamplesFW)
      |     if ~strcmp(u16NSamplesFW_bkup,'0')
      |       set_param(gcb,'u16NSamplesFW','0');
      |     end
      |   else
      |     tmps=num2str(u16NSamplesFW);
      |     if ~strcmp(u16NSamplesFW_bkup,tmps)
      |       set_param(gcb,'u16NSamplesFW',tmps);
      |     end
      |   end
      |   if isnan(f16PropGainQ)
      |     if ~strcmp(f16PropGainQ_bkup,'0')
      |       set_param(gcb,'f16PropGainQ','0');
      |     end
      |   else
      |     tmps=num2str(f16PropGainQ);
      |     if ~strcmp(f16PropGainQ_bkup,tmps)
      |       set_param(gcb,'f16PropGainQ',tmps);
      |     end
      |   end
      |   if isnan(f16IntegGainQ)
      |     if ~strcmp(f16IntegGainQ_bkup,'0')
      |       set_param(gcb,'f16IntegGainQ','0');
      |     end
      |   else
      |     tmps=num2str(f16IntegGainQ);
      |     if ~strcmp(f16IntegGainQ_bkup,tmps)
      |       set_param(gcb,'f16IntegGainQ',tmps);
      |     end
      |   end
      |   if isnan(s16PropGainShiftQ)
      |     if ~strcmp(s16PropGainShiftQ_bkup,'0')
      |       set_param(gcb,'s16PropGainShiftQ','0');
      |     end
      |   else
      |     tmps=num2str(s16PropGainShiftQ);
      |     if ~strcmp(s16PropGainShiftQ_bkup,tmps)
      |       set_param(gcb,'s16PropGainShiftQ',tmps);
      |     end
      |   end
      |   if isnan(s16IntegGainShiftQ)
      |     if ~strcmp(s16IntegGainShiftQ_bkup,'0')
      |       set_param(gcb,'s16IntegGainShiftQ','0');
      |     end
      |   else
      |     tmps=num2str(s16IntegGainShiftQ);
      |     if ~strcmp(s16IntegGainShiftQ_bkup,tmps)
      |       set_param(gcb,'s16IntegGainShiftQ',tmps);
      |     end
      |   end
      |   if isnan(f16LowerLimitQ)
      |     if ~strcmp(f16LowerLimitQ_bkup,'0')
      |       set_param(gcb,'f16LowerLimitQ','0');
      |     end
      |   else
      |     tmps=num2str(f16LowerLimitQ);
      |     if ~strcmp(f16LowerLimitQ_bkup,tmps)
      |       set_param(gcb,'f16LowerLimitQ',tmps);
      |     end
      |   end
      |   if isnan(f16UpperLimitQ)
      |     if ~strcmp(f16UpperLimitQ_bkup,'0')
      |       set_param(gcb,'f16UpperLimitQ','0');
      |     end
      |   else
      |     tmps=num2str(f16UpperLimitQ);
      |     if ~strcmp(f16UpperLimitQ_bkup,tmps)
      |       set_param(gcb,'f16UpperLimitQ',tmps);
      |     end
      |   end
      |   if isnan(f16PropGainFW)
      |     if ~strcmp(f16PropGainFW_bkup,'0')
      |       set_param(gcb,'f16PropGainFW','0');
      |     end
      |   else
      |     tmps=num2str(f16PropGainFW);
      |     if ~strcmp(f16PropGainFW_bkup,tmps)
      |       set_param(gcb,'f16PropGainFW',tmps);
      |     end
      |   end
      |   if isnan(f16IntegGainFW)
      |     if ~strcmp(f16IntegGainFW_bkup,'0')
      |       set_param(gcb,'f16IntegGainFW','0');
      |     end
      |   else
      |     tmps=num2str(f16IntegGainFW);
      |     if ~strcmp(f16IntegGainFW_bkup,tmps)
      |       set_param(gcb,'f16IntegGainFW',tmps);
      |     end
      |   end
      |   if isnan(s16PropGainShiftFW)
      |     if ~strcmp(s16PropGainShiftFW_bkup,'0')
      |       set_param(gcb,'s16PropGainShiftFW','0');
      |     end
      |   else
      |     tmps=num2str(s16PropGainShiftFW);
      |     if ~strcmp(s16PropGainShiftFW_bkup,tmps)
      |       set_param(gcb,'s16PropGainShiftFW',tmps);
      |     end
      |   end
      |   if isnan(s16IntegGainShiftFW)
      |     if ~strcmp(s16IntegGainShiftFW_bkup,'0')
      |       set_param(gcb,'s16IntegGainShiftFW','0');
      |     end
      |   else
      |     tmps=num2str(s16IntegGainShiftFW);
      |     if ~strcmp(s16IntegGainShiftFW_bkup,tmps)
      |       set_param(gcb,'s16IntegGainShiftFW',tmps);
      |     end
      |   end
      |   if isnan(f16LowerLimitFW)
      |     if ~strcmp(f16LowerLimitFW_bkup,'0')
      |       set_param(gcb,'f16LowerLimitFW','0');
      |     end
      |   else
      |     tmps=num2str(f16LowerLimitFW);
      |     if ~strcmp(f16LowerLimitFW_bkup,tmps)
      |       set_param(gcb,'f16LowerLimitFW',tmps);
      |     end
      |   end
      |   if isnan(f16UpperLimitFW)
      |     if ~strcmp(f16UpperLimitFW_bkup,'0')
      |       set_param(gcb,'f16UpperLimitFW','0');
      |     end
      |   else
      |     tmps=num2str(f16UpperLimitFW);
      |     if ~strcmp(f16UpperLimitFW_bkup,tmps)
      |       set_param(gcb,'f16UpperLimitFW',tmps);
      |     end
      |   end
      |   if isnan(f32RampUp)
      |     if ~strcmp(f32RampUp_bkup,'0')
      |       set_param(gcb,'f32RampUp','0');
      |     end
      |   else
      |     tmps=num2str(f32RampUp);
      |     if ~strcmp(f32RampUp_bkup,tmps)
      |       set_param(gcb,'f32RampUp',tmps);
      |     end
      |   end
      |   if isnan(f32RampDown)
      |     if ~strcmp(f32RampDown_bkup,'0')
      |       set_param(gcb,'f32RampDown','0');
      |     end
      |   else
      |     tmps=num2str(f32RampDown);
      |     if ~strcmp(f32RampDown_bkup,tmps)
      |       set_param(gcb,'f32RampDown',tmps);
      |     end
      |   end
      | end
      mask prompts: showStates "Show internal states:"; resetStatesEnable "Internal state after reset:"; showDebugOutputs "Show debugging outputs:"; f32State_Out_showOutput "Output speed ramp state (f32State_Out)"; SampleTime "Sample time (-1 for inherited):"; wf0 "Speed loop natural frequency f0 [Hz]:"; wksi "Speed loop attenuation ξ:"; J "Moment of inertia J [kg*m^2]:"; Kt "Motor torque constant Kt [N*m/A]:"; lambdaW "Speed MA filter smoothing factor λ (0..1):"; lambdaFW "Field weakening MA filter smoothing factor λ (0..1):"; Idmax "Maximum negative d-axis current (demagnetization current - CAUTION!) [A]:"; ramprpm "Speed ramp slope [ΔRPM per speed loop iteration]:"; mechspeed "Maximum mechanical speed of the motor [RPM]:"; polepairs "Number of pole pairs of the motor:"; uscale "U_max (maximum DC bus voltage) [V]:"; iscale "I_max (maximum phase current) [A]:"; autoCalcEn "Calculate implementation parameters from physical parameters"; u16NSamplesW "u16NSamplesW (velocity GDFLIB_FilterMA - recalculated smoothing factor):"; u16NSamplesFW "u16NSamplesFW (FW GDFLIB_FilterMA - recalculated smoothing factor):"; f16PropGainQ "f16PropGainQ (q-axis GFLIB_ControllerPIpAW - proportional gain):"; f16IntegGainQ "f16IntegGainQ (q-axis GFLIB_ControllerPIpAW - integral gain):"; s16PropGainShiftQ "s16PropGainShiftQ (q-axis GFLIB_ControllerPIpAW - scaling bitwise shift applied to the proportional gain):"; s16IntegGainShiftQ "s16IntegGainShiftQ (q-axis GFLIB_ControllerPIpAW - scaling bitwise shift applied to the integral gain):"; f16LowerLimitQ "f16LowerLimitQ (q-axis GFLIB_ControllerPIpAW - lower limit):"; f16UpperLimitQ "f16UpperLimitQ (q-axis GFLIB_ControllerPIpAW - upper limit):"; f16PropGainFW "f16PropGainFW (FW GFLIB_ControllerPIpAW - proportional gain):"; f16IntegGainFW "f16IntegGainFW (FW GFLIB_ControllerPIpAW - integral gain):"; s16PropGainShiftFW "s16PropGainShiftFW (FW GFLIB_ControllerPIpAW - scaling bitwise shift applied to the proportional gain):"; s16IntegGainShiftFW "s16IntegGainShiftFW (FW GFLIB_ControllerPIpAW - scaling bitwise shift applied to the integral gain):"; f16LowerLimitFW "f16LowerLimitFW (FW GFLIB_ControllerPIpAW - lower limit):"; f16UpperLimitFW "f16UpperLimitFW (FW GFLIB_ControllerPIpAW - upper limit):"; f32RampUp "f32RampUp (Ramp up increment coefficient):"; f32RampDown "f32RampDown (Ramp decrement coefficient):"; SampleTime_1 "Discrete sample time:"
      mask help: Speed loop controller with Field Weakening capability for the PMSM field-oriented control algorithm in 16-bit fixed-point fractional implementation. This block supports re-initialization of the internal state during simulation. If the block is reset, the outputs of the MA filters, PI controllers, and the ramp will be aligned with the inputs f16FilterMAWOut_preset, f16FilterMAFWOut_preset, f16ControllerPIpAWQOut_preset, f16ControllerPIpAWFWOut_preset, and f32RampOut_preset. Refer to the AMMCLIB User's Guide for further details.
      mask init:
      | ddName = get_param(bdroot,'DataDictionary');
      | if length(ddName)==0
      |   set_param(bdroot,'DataDictionary','ammclib_types.sldd');
      | else
      |   dd = Simulink.data.dictionary.open(ddName);
      |   data = getSection(dd,'Design Data');
      |   if ~exist(data,'SWLIBS_2Syst_F16')
      |     addDataSource(dd,'ammclib_types.sldd');
      |     saveChanges(dd);
      |   end
      | end
      | outputsChanged = 0;
      | 
      | if showStates == 1
      |   % hidden state variables
      |   if strcmp(get_param([gcb '/u16NSamplesW'], 'BlockType'), 'Inport')
      |     posblk = get_param(gcb, 'Position');
      | 
      |     pos = get_param([gcb, '/u16NSamplesW'], 'Position');
      |     orient = get_param([gcb, '/u16NSamplesW'], 'Orientation');
      |     delete_block([gcb, '/u16NSamplesW']);
      |     add_block('built-in/Ground', [gcb, '/u16NSamplesW'], 'Position', pos, 'Orientation', orient);
      | 
      |     pos = get_param([gcb, '/u16NSamplesFW'], 'Position');
      |     orient = get_param([gcb, '/u16NSamplesFW'], 'Orientation');
      |     delete_block([gcb, '/u16NSamplesFW']);
      |     add_block('built-in/Ground', [gcb, '/u16NSamplesFW'], 'Position', pos, 'Orientation', orient);
      | 
      |     pos = get_param([gcb, '/f16PropGainQ'], 'Position');
      |     orient = get_param([gcb, '/f16PropGainQ'], 'Orientation');
      |     delete_block([gcb, '/f16PropGainQ']);
      |     add_block('built-in/Ground', [gcb, '/f16PropGainQ'], 'Position', pos, 'Orientation', orient);
      | 
      |     pos = get_param([gcb, '/f16IntegGainQ'], 'Position');
      |     orient = get_param([gcb, '/f16IntegGainQ'], 'Orientation');
      |     delete_block([gcb, '/f16IntegGainQ']);
      |     add_block('built-in/Ground', [gcb, '/f16IntegGainQ'], 'Position', pos, 'Orientation', orient);
      | 
      |     pos = get_param([gcb, '/s16PropGainShiftQ'], 'Position');
      |     orient = get_param([gcb, '/s16PropGainShiftQ'], 'Orientation');
      |     delete_block([gcb, '/s16PropGainShiftQ']);
      |     add_block('built-in/Ground', [gcb, '/s16PropGainShiftQ'], 'Position', pos, 'Orientation', orient);
      | 
      |     pos = get_param([gcb, '/s16IntegGainShiftQ'], 'Position');
      |     orient = get_param([gcb, '/s16IntegGainShiftQ'], 'Orientation');
      |     delete_block([gcb, '/s16IntegGainShiftQ']);
      |     add_block('built-in/Ground', [gcb, '/s16IntegGainShiftQ'], 'Position', pos, 'Orientation', orient);
      | 
      |     pos = get_param([gcb, '/f16LowerLimitQ'], 'Position');
      |     orient = get_param([gcb, '/f16LowerLimitQ'], 'Orientation');
      |     delete_block([gcb, '/f16LowerLimitQ']);
      |     add_block('built-in/Ground', [gcb, '/f16LowerLimitQ'], 'Position', pos, 'Orientation', orient);
      | 
      |     pos = get_param([gcb, '/f16UpperLimitQ'], 'Position');
      |     orient = get_param([gcb, '/f16UpperLimitQ'], 'Orientation');
      |     delete_block([gcb, '/f16UpperLimitQ']);
      |     add_block('built-in/Ground', [gcb, '/f16UpperLimitQ'], 'Position', pos, 'Orientation', orient);
      | 
      |     pos = get_param([gcb, '/f16PropGainFW'], 'Position');
      |     orient = get_param([gcb, '/f16PropGainFW'], 'Orientation');
      |     delete_block([gcb, '/f16PropGainFW']);
      |     add_block('built-in/Ground', [gcb, '/f16PropGainFW'], 'Position', pos, 'Orientation', orient);
      | 
      |     pos = get_param([gcb, '/f16IntegGainFW'], 'Position');
      |     orient = get_param([gcb, '/f16IntegGainFW'], 'Orientation');
      |     delete_block([gcb, '/f16IntegGainFW']);
      |     add_block('built-in/Ground', [gcb, '/f16IntegGainFW'], 'Position', pos, 'Orientation', orient);
      | 
      |     pos = get_param([gcb, '/s16PropGainShiftFW'], 'Position');
      |     orient = get_param([gcb, '/s16PropGainShiftFW'], 'Orientation');
      |     delete_block([gcb, '/s16PropGainShiftFW']);
      |     add_block('built-in/Ground', [gcb, '/s16PropGainShiftFW'], 'Position', pos, 'Orientation', orient);
      | 
      |     pos = get_param([gcb, '/s16IntegGainShiftFW'], 'Position');
      |     orient = get_param([gcb, '/s16IntegGainShiftFW'], 'Orientation');
      |     delete_block([gcb, '/s16IntegGainShiftFW']);
      |     add_block('built-in/Ground', [gcb, '/s16IntegGainShiftFW'], 'Position', pos, 'Orientation', orient);
      | 
      |     pos = get_param([gcb, '/f16LowerLimitFW'], 'Position');
      |     orient = get_param([gcb, '/f16LowerLimitFW'], 'Orientation');
      |     delete_block([gcb, '/f16LowerLimitFW']);
      |     add_block('built-in/Ground', [gcb, '/f16LowerLimitFW'], 'Position', pos, 'Orientation', orient);
      | 
      |     pos = get_param([gcb, '/f16UpperLimitFW'], 'Position');
      |     orient = get_param([gcb, '/f16UpperLimitFW'], 'Orientation');
      |     delete_block([gcb, '/f16UpperLimitFW']);
      |     add_block('built-in/Ground', [gcb, '/f16UpperLimitFW'], 'Position', pos, 'Orientation', orient);
      | 
      |     pos = get_param([gcb, '/f32RampUp'], 'Position');
      |     orient = get_param([gcb, '/f32RampUp'], 'Orientation');
      |     delete_block([gcb, '/f32RampUp']);
      |     add_block('built-in/Ground', [gcb, '/f32RampUp'], 'Position', pos, 'Orientation', orient);
      | 
      |     pos = get_param([gcb, '/f32RampDown'], 'Position');
      |     orient = get_param([gcb, '/f32RampDown'], 'Orientation');
      |     delete_block([gcb, '/f32RampDown']);
      |     add_block('built-in/Ground', [gcb, '/f32RampDown'], 'Position', pos, 'Orientation', orient);
      | 
      |     pos = get_param([gcb, '/f16IQReqK_1'], 'Position');
      |     orient = get_param([gcb, '/f16IQReqK_1'], 'Orientation');
      |     delete_block([gcb, '/f16IQReqK_1']);
      |     add_block('built-in/Ground', [gcb, '/f16IQReqK_1'], 'Position', pos, 'Orientation', orient);
      | 
      |     pos = get_param([gcb, '/f32AccW'], 'Position');
      |     orient = get_param([gcb, '/f32AccW'], 'Orientation');
      |     delete_block([gcb, '/f32AccW']);
      |     add_block('built-in/Ground', [gcb, '/f32AccW'], 'Position', pos, 'Orientation', orient);
      | 
      |     pos = get_param([gcb, '/f32AccFW'], 'Position');
      |     orient = get_param([gcb, '/f32AccFW'], 'Orientation');
      |     delete_block([gcb, '/f32AccFW']);
      |     add_block('built-in/Ground', [gcb, '/f32AccFW'], 'Position', pos, 'Orientation', orient);
      | 
      |     pos = get_param([gcb, '/f32IntegPartK_1Q'], 'Position');
      |     orient = get_param([gcb, '/f32IntegPartK_1Q'], 'Orientation');
      |     delete_block([gcb, '/f32IntegPartK_1Q']);
      |     add_block('built-in/Ground', [gcb, '/f32IntegPartK_1Q'], 'Position', pos, 'Orientation', orient);
      | 
      |     pos = get_param([gcb, '/f16InK_1Q'], 'Position');
      |     orient = get_param([gcb, '/f16InK_1Q'], 'Orientation');
      |     delete_block([gcb, '/f16InK_1Q']);
      |     add_block('built-in/Ground', [gcb, '/f16InK_1Q'], 'Position', pos, 'Orientation', orient);
      | 
      |     pos = get_param([gcb, '/f32IntegPartK_1FW'], 'Position');
      |     orient = get_param([gcb, '/f32IntegPartK_1FW'], 'Orientation');
      |     delete_block([gcb, '/f32IntegPartK_1FW']);
      |     add_block('built-in/Ground', [gcb, '/f32IntegPartK_1FW'], 'Position', pos, 'Orientation', orient);
      | 
      |     pos = get_param([gcb, '/f16InK_1FW'], 'Position');
      |     orient = get_param([gcb, '/f16InK_1FW'], 'Orientation');
      |     delete_block([gcb, '/f16InK_1FW']);
      |     add_block('built-in/Ground', [gcb, '/f16InK_1FW'], 'Position', pos, 'Orientation', orient);
      | 
      |     pos = get_param([gcb, '/f32State'], 'Position');
      |     orient = get_param([gcb, '/f32State'], 'Orientation');
      |     delete_block([gcb, '/f32State']);
      |     add_block('built-in/Ground', [gcb, '/f32State'], 'Position', pos, 'Orientation', orient);
      | 
      | 
      |     pmask=Simulink.Mask.get(gcb);
      |     pctrl=pmask.getParameter('SampleTime');
      |     pctrl.set('TypeOptions',{'f16VelocityReq/SampleTime','f16VelocityFbck/SampleTime','f16IQFbck/SampleTime','f16UQReq/SampleTime','f16UQLim/SampleTime','f16FilterMAWOut_preset/SampleTime','f16FilterMAFWOut_preset/SampleTime','f16ControllerPIpAWQOut_preset/SampleTime','f16ControllerPIpAWFWOut_preset/SampleTime','f32RampOut_preset/SampleTime'});
      | 
      |     pos = get_param([gcb '/f32AccW_Out'], 'Position');
      |     orient = get_param([gcb '/f32AccW_Out'], 'Orientation');
      |     delete_block([gcb '/f32AccW_Out']);
      |     add_block('built-in/Terminator', [gcb '/f32AccW_Out'], 'Position', pos, 'Orientation', orient);
      | 
      |     pos = get_param([gcb '/f32AccFW_Out'], 'Position');
      |     orient = get_param([gcb '/f32AccFW_Out'], 'Orientation');
      |     delete_block([gcb '/f32AccFW_Out']);
      |     add_block('built-in/Terminator', [gcb '/f32AccFW_Out'], 'Position', pos, 'Orientation', orient);
      | 
      |     pos = get_param([gcb '/f32IntegPartK_1Q_Out'], 'Position');
      |     orient = get_param([gcb '/f32IntegPartK_1Q_Out'], 'Orientation');
      |     delete_block([gcb '/f32IntegPartK_1Q_Out']);
      |     add_block('built-in/Terminator', [gcb '/f32IntegPartK_1Q_Out'], 'Position', pos, 'Orientation', orient);
      | 
      |     pos = get_param([gcb '/f16InK_1Q_Out'], 'Position');
      |     orient = get_param([gcb '/f16InK_1Q_Out'], 'Orientation');
      |     delete_block([gcb '/f16InK_1Q_Out']);
      |     add_block('built-in/Terminator', [gcb '/f16InK_1Q_Out'], 'Position', pos, 'Orientation', orient);
      | 
      |     pos = get_param([gcb '/f32IntegPartK_1FW_Out'], 'Position');
      |     orient = get_param([gcb '/f32IntegPartK_1FW_Out'], 'Orientation');
      |     delete_block([gcb '/f32IntegPartK_1FW_Out']);
      |     add_block('built-in/Terminator', [gcb '/f32IntegPartK_1FW_Out'], 'Position', pos, 'Orientation', orient);
      | 
      |     pos = get_param([gcb '/f16InK_1FW_Out'], 'Position');
      |     orient = get_param([gcb '/f16InK_1FW_Out'], 'Orientation');
      |     delete_block([gcb '/f16InK_1FW_Out']);
      |     add_block('built-in/Terminator', [gcb '/f16InK_1FW_Out'], 'Position', pos, 'Orientation', orient);
      | 
      |     if strcmp(get_param([gcb '/f16WReqFilt'], 'BlockType'), 'Outport')
      |       pos = get_param([gcb '/f16WReqFilt'], 'Position');
      |       orient = get_param([gcb '/f16WReqFilt'], 'Orientation');
      |       delete_block([gcb '/f16WReqFilt']);
      |       add_block('built-in/Terminator', [gcb '/f16WReqFilt'], 'Position', pos, 'Orientation', orient);
      | 
      |       pos = get_param([gcb '/f16WErr'], 'Position');
      |       orient = get_param([gcb '/f16WErr'], 'Orientation');
      |       delete_block([gcb '/f16WErr']);
      |       add_block('built-in/Terminator', [gcb '/f16WErr'], 'Position', pos, 'Orientation', orient);
      | 
      |       pos = get_param([gcb '/f16IDQReqAmp'], 'Position');
      |       orient = get_param([gcb '/f16IDQReqAmp'], 'Orientation');
      |       delete_block([gcb '/f16IDQReqAmp']);
      |       add_block('built-in/Terminator', [gcb '/f16IDQReqAmp'], 'Position', pos, 'Orientation', orient);
      | 
      |       pos = get_param([gcb '/f16WFbckFilt'], 'Position');
      |       orient = get_param([gcb '/f16WFbckFilt'], 'Orientation');
      |       delete_block([gcb '/f16WFbckFilt']);
      |       add_block('built-in/Terminator', [gcb '/f16WFbckFilt'], 'Position', pos, 'Orientation', orient);
      | 
      |       pos = get_param([gcb '/f16IQErrSign'], 'Position');
      |       orient = get_param([gcb '/f16IQErrSign'], 'Orientation');
      |       delete_block([gcb '/f16IQErrSign']);
      |       add_block('built-in/Terminator', [gcb '/f16IQErrSign'], 'Position', pos, 'Orientation', orient);
      | 
      |       pos = get_param([gcb '/f16IQErr'], 'Position');
      |       orient = get_param([gcb '/f16IQErr'], 'Orientation');
      |       delete_block([gcb '/f16IQErr']);
      |       add_block('built-in/Terminator', [gcb '/f16IQErr'], 'Position', pos, 'Orientation', orient);
      | 
      |       pos = get_param([gcb '/f16FWErr'], 'Position');
      |       orient = get_param([gcb '/f16FWErr'], 'Orientation');
      |       delete_block([gcb '/f16FWErr']);
      |       add_block('built-in/Terminator', [gcb '/f16FWErr'], 'Position', pos, 'Orientation', orient);
      | 
      |       pos = get_param([gcb '/f16UQErr'], 'Position');
      |       orient = get_param([gcb '/f16UQErr'], 'Orientation');
      |       delete_block([gcb '/f16UQErr']);
      |       add_block('built-in/Terminator', [gcb '/f16UQErr'], 'Position', pos, 'Orientation', orient);
      | 
      |       pos = get_param([gcb '/f16FWErrFilt'], 'Position');
      |       orient = get_param([gcb '/f16FWErrFilt'], 'Orientation');
      |       delete_block([gcb '/f16FWErrFilt']);
      |       add_block('built-in/Terminator', [gcb '/f16FWErrFilt'], 'Position', pos, 'Orientation', orient);
      | 
      |       pos = get_param([gcb '/f16FWAngle'], 'Position');
      |       orient = get_param([gcb '/f16FWAngle'], 'Orientation');
      |       delete_block([gcb '/f16FWAngle']);
      |       add_block('built-in/Terminator', [gcb '/f16FWAngle'], 'Position', pos, 'Orientation', orient);
      | 
      |       pos = get_param([gcb '/f16FWSin'], 'Position');
      |       orient = get_param([gcb '/f16FWSin'], 'Orientation');
      |       delete_block([gcb '/f16FWSin']);
      |       add_block('built-in/Terminator', [gcb '/f16FWSin'], 'Position', pos, 'Orientation', orient);
      | 
      |       pos = get_param([gcb '/f16FWCos'], 'Position');
      |       orient = get_param([gcb '/f16FWCos'], 'Orientation');
      |       delete_block([gcb '/f16FWCos']);
      |       add_block('built-in/Terminator', [gcb '/f16FWCos'], 'Position', pos, 'Orientation', orient);
      | 
      |     end
      | 
      |     set_param([gcb '/f16VelocityReq'], 'Port', '1');
      |     set_param([gcb '/f16VelocityFbck'], 'Port', '2');
      |     set_param([gcb '/f16IQFbck'], 'Port', '3');
      |     set_param([gcb '/f16UQReq'], 'Port', '4');
      |     set_param([gcb '/f16UQLim'], 'Port', '5');
      |     set_param([gcb '/f16FilterMAWOut_preset'], 'Port', '6');
      |     set_param([gcb '/f16FilterMAFWOut_preset'], 'Port', '7');
      |     set_param([gcb '/f16ControllerPIpAWQOut_preset'], 'Port', '8');
      |     set_param([gcb '/f16ControllerPIpAWFWOut_preset'], 'Port', '9');
      |     set_param([gcb '/f32RampOut_preset'], 'Port', '10');
      | 
      |     tmpOutCnt=0;
      |     tmpOutCnt=tmpOutCnt+1;
      |     set_param([gcb '/pIDQReq'], 'Port', num2str(tmpOutCnt));
      |     tmpOutCnt=tmpOutCnt+1;
      |     set_param([gcb '/u16LimitFlagQ'], 'Port', num2str(tmpOutCnt));
      |     tmpOutCnt=tmpOutCnt+1;
      |     set_param([gcb '/u16LimitFlagFW'], 'Port', num2str(tmpOutCnt));
      |     if strcmp(get_param([gcb '/f32State_Out'], 'BlockType'), 'Outport')
      |       tmpOutCnt=tmpOutCnt+1;
      |       set_param([gcb '/f32State_Out'], 'Port', num2str(tmpOutCnt));
      |     end
      | 
      |   autoCalcEn=get_param(gcb,'autoCalcEn');
      |   if strcmp(autoCalcEn,'on')
      |     set_param(gcb,'MaskEnables',{'on','on','off','on','on','on','on','on','on','on','on','on','on','on','on','on','on','on','on','on','on','on','on','on','on','on','on','on','on','on','on','on','on','on','off'});
      |   else
      |     set_param(gcb,'MaskEnables',{'on','on','off','on','on','off','off','off','off','off','off','off','off','off','off','off','off','on','on','on','on','on','on','on','on','on','on','on','on','on','on','on','on','on','off'});
      |   end
      | 
      |     if (posblk(4) - posblk(2)) > 275
      |       height = 275;
      |       set_param(gcb,'Position',[posblk(1), posblk(2), posblk(3), posblk(2)+height])
      |     end
      |   end
      | else
      |   % shown state variables
      |   if strcmp(get_param([gcb '/u16NSamplesW'], 'BlockType'), 'Ground')
      |     posblk = get_param(gcb, 'Position');
      | 
      |     pos = get_param([gcb, '/u16NSamplesW'], 'Position');
      |     orient = get_param([gcb, '/u16NSamplesW'], 'Orientation');
      |     delete_block([gcb, '/u16NSamplesW']);
      |     add_block('built-in/Inport', [gcb, '/u16NSamplesW'], 'Position', pos, 'Orientation', orient, 'OutDataTypeStr', 'uint16');
      | 
      |     pos = get_param([gcb, '/u16NSamplesFW'], 'Position');
      |     orient = get_param([gcb, '/u16NSamplesFW'], 'Orientation');
      |     delete_block([gcb, '/u16NSamplesFW']);
      |     add_block('built-in/Inport', [gcb, '/u16NSamplesFW'], 'Position', pos, 'Orientation', orient, 'OutDataTypeStr', 'uint16');
      | 
      |     pos = get_param([gcb, '/f16PropGainQ'], 'Position');
      |     orient = get_param([gcb, '/f16PropGainQ'], 'Orientation');
      |     delete_block([gcb, '/f16PropGainQ']);
      |     add_block('built-in/Inport', [gcb, '/f16PropGainQ'], 'Position', pos, 'Orientation', orient, 'OutDataTypeStr', 'int16');
      | 
      |     pos = get_param([gcb, '/f16IntegGainQ'], 'Position');
      |     orient = get_param([gcb, '/f16IntegGainQ'], 'Orientation');
      |     delete_block([gcb, '/f16IntegGainQ']);
      |     add_block('built-in/Inport', [gcb, '/f16IntegGainQ'], 'Position', pos, 'Orientation', orient, 'OutDataTypeStr', 'int16');
      | 
      |     pos = get_param([gcb, '/s16PropGainShiftQ'], 'Position');
      |     orient = get_param([gcb, '/s16PropGainShiftQ'], 'Orientation');
      |     delete_block([gcb, '/s16PropGainShiftQ']);
      |     add_block('built-in/Inport', [gcb, '/s16PropGainShiftQ'], 'Position', pos, 'Orientation', orient, 'OutDataTypeStr', 'int16');
      | 
      |     pos = get_param([gcb, '/s16IntegGainShiftQ'], 'Position');
      |     orient = get_param([gcb, '/s16IntegGainShiftQ'], 'Orientation');
      |     delete_block([gcb, '/s16IntegGainShiftQ']);
      |     add_block('built-in/Inport', [gcb, '/s16IntegGainShiftQ'], 'Position', pos, 'Orientation', orient, 'OutDataTypeStr', 'int16');
      | 
      |     pos = get_param([gcb, '/f16LowerLimitQ'], 'Position');
      |     orient = get_param([gcb, '/f16LowerLimitQ'], 'Orientation');
      |     delete_block([gcb, '/f16LowerLimitQ']);
      |     add_block('built-in/Inport', [gcb, '/f16LowerLimitQ'], 'Position', pos, 'Orientation', orient, 'OutDataTypeStr', 'int16');
      | 
      |     pos = get_param([gcb, '/f16UpperLimitQ'], 'Position');
      |     orient = get_param([gcb, '/f16UpperLimitQ'], 'Orientation');
      |     delete_block([gcb, '/f16UpperLimitQ']);
      |     add_block('built-in/Inport', [gcb, '/f16UpperLimitQ'], 'Position', pos, 'Orientation', orient, 'OutDataTypeStr', 'int16');
      | 
      |     pos = get_param([gcb, '/f16PropGainFW'], 'Position');
      |     orient = get_param([gcb, '/f16PropGainFW'], 'Orientation');
      |     delete_block([gcb, '/f16PropGainFW']);
      |     add_block('built-in/Inport', [gcb, '/f16PropGainFW'], 'Position', pos, 'Orientation', orient, 'OutDataTypeStr', 'int16');
      | 
      |     pos = get_param([gcb, '/f16IntegGainFW'], 'Position');
      |     orient = get_param([gcb, '/f16IntegGainFW'], 'Orientation');
      |     delete_block([gcb, '/f16IntegGainFW']);
      |     add_block('built-in/Inport', [gcb, '/f16IntegGainFW'], 'Position', pos, 'Orientation', orient, 'OutDataTypeStr', 'int16');
      | 
      |     pos = get_param([gcb, '/s16PropGainShiftFW'], 'Position');
      |     orient = get_param([gcb, '/s16PropGainShiftFW'], 'Orientation');
      |     delete_block([gcb, '/s16PropGainShiftFW']);
      |     add_block('built-in/Inport', [gcb, '/s16PropGainShiftFW'], 'Position', pos, 'Orientation', orient, 'OutDataTypeStr', 'int16');
      | 
      |     pos = get_param([gcb, '/s16IntegGainShiftFW'], 'Position');
      |     orient = get_param([gcb, '/s16IntegGainShiftFW'], 'Orientation');
      |     delete_block([gcb, '/s16IntegGainShiftFW']);
      |     add_block('built-in/Inport', [gcb, '/s16IntegGainShiftFW'], 'Position', pos, 'Orientation', orient, 'OutDataTypeStr', 'int16');
      | 
      |     pos = get_param([gcb, '/f16LowerLimitFW'], 'Position');
      |     orient = get_param([gcb, '/f16LowerLimitFW'], 'Orientation');
      |     delete_block([gcb, '/f16LowerLimitFW']);
      |     add_block('built-in/Inport', [gcb, '/f16LowerLimitFW'], 'Position', pos, 'Orientation', orient, 'OutDataTypeStr', 'int16');
      | 
      |     pos = get_param([gcb, '/f16UpperLimitFW'], 'Position');
      |     orient = get_param([gcb, '/f16UpperLimitFW'], 'Orientation');
      |     delete_block([gcb, '/f16UpperLimitFW']);
      |     add_block('built-in/Inport', [gcb, '/f16UpperLimitFW'], 'Position', pos, 'Orientation', orient, 'OutDataTypeStr', 'int16');
      | 
      |     pos = get_param([gcb, '/f32RampUp'], 'Position');
      |     orient = get_param([gcb, '/f32RampUp'], 'Orientation');
      |     delete_block([gcb, '/f32RampUp']);
      |     add_block('built-in/Inport', [gcb, '/f32RampUp'], 'Position', pos, 'Orientation', orient, 'OutDataTypeStr', 'int32');
      | 
      |     pos = get_param([gcb, '/f32RampDown'], 'Position');
      |     orient = get_param([gcb, '/f32RampDown'], 'Orientation');
      |     delete_block([gcb, '/f32RampDown']);
      |     add_block('built-in/Inport', [gcb, '/f32RampDown'], 'Position', pos, 'Orientation', orient, 'OutDataTypeStr', 'int32');
      | 
      |     pos = get_param([gcb, '/f16IQReqK_1'], 'Position');
      |     orient = get_param([gcb, '/f16IQReqK_1'], 'Orientation');
      |     delete_block([gcb, '/f16IQReqK_1']);
      |     add_block('built-in/Inport', [gcb, '/f16IQReqK_1'], 'Position', pos, 'Orientation', orient, 'OutDataTypeStr', 'int16');
      | 
      |     pos = get_param([gcb, '/f32AccW'], 'Position');
      |     orient = get_param([gcb, '/f32AccW'], 'Orientation');
      |     delete_block([gcb, '/f32AccW']);
      |     add_block('built-in/Inport', [gcb, '/f32AccW'], 'Position', pos, 'Orientation', orient, 'OutDataTypeStr', 'int32');
      | 
      |     pos = get_param([gcb, '/f32AccFW'], 'Position');
      |     orient = get_param([gcb, '/f32AccFW'], 'Orientation');
      |     delete_block([gcb, '/f32AccFW']);
      |     add_block('built-in/Inport', [gcb, '/f32AccFW'], 'Position', pos, 'Orientation', orient, 'OutDataTypeStr', 'int32');
      | 
      |     pos = get_param([gcb, '/f32IntegPartK_1Q'], 'Position');
      |     orient = get_param([gcb, '/f32IntegPartK_1Q'], 'Orientation');
      |     delete_block([gcb, '/f32IntegPartK_1Q']);
      |     add_block('built-in/Inport', [gcb, '/f32IntegPartK_1Q'], 'Position', pos, 'Orientation', orient, 'OutDataTypeStr', 'int32');
      | 
      |     pos = get_param([gcb, '/f16InK_1Q'], 'Position');
      |     orient = get_param([gcb, '/f16InK_1Q'], 'Orientation');
      |     delete_block([gcb, '/f16InK_1Q']);
      |     add_block('built-in/Inport', [gcb, '/f16InK_1Q'], 'Position', pos, 'Orientation', orient, 'OutDataTypeStr', 'int16');
      | 
      |     pos = get_param([gcb, '/f32IntegPartK_1FW'], 'Position');
      |     orient = get_param([gcb, '/f32IntegPartK_1FW'], 'Orientation');
      |     delete_block([gcb, '/f32IntegPartK_1FW']);
      |     add_block('built-in/Inport', [gcb, '/f32IntegPartK_1FW'], 'Position', pos, 'Orientation', orient, 'OutDataTypeStr', 'int32');
      | 
      |     pos = get_param([gcb, '/f16InK_1FW'], 'Position');
      |     orient = get_param([gcb, '/f16InK_1FW'], 'Orientation');
      |     delete_block([gcb, '/f16InK_1FW']);
      |     add_block('built-in/Inport', [gcb, '/f16InK_1FW'], 'Position', pos, 'Orientation', orient, 'OutDataTypeStr', 'int16');
      | 
      |     pos = get_param([gcb, '/f32State'], 'Position');
      |     orient = get_param([gcb, '/f32State'], 'Orientation');
      |     delete_block([gcb, '/f32State']);
      |     add_block('built-in/Inport', [gcb, '/f32State'], 'Position', pos, 'Orientation', orient, 'OutDataTypeStr', 'int32');
      | 
      | 
      | 
      |     pos = get_param([gcb '/f32AccW_Out'], 'Position');
      |     orient = get_param([gcb '/f32AccW_Out'], 'Orientation');
      |     delete_block([gcb '/f32AccW_Out']);
      |     add_block('built-in/Outport', [gcb '/f32AccW_Out'], 'Position', pos, 'Orientation', orient);
      | 
      |     pos = get_param([gcb '/f32AccFW_Out'], 'Position');
      |     orient = get_param([gcb '/f32AccFW_Out'], 'Orientation');
      |     delete_block([gcb '/f32AccFW_Out']);
      |     add_block('built-in/Outport', [gcb '/f32AccFW_Out'], 'Position', pos, 'Orientation', orient);
      | 
      |     pos = get_param([gcb '/f32IntegPartK_1Q_Out'], 'Position');
      |     orient = get_param([gcb '/f32IntegPartK_1Q_Out'], 'Orientation');
      |     delete_block([gcb '/f32IntegPartK_1Q_Out']);
      |     add_block('built-in/Outport', [gcb '/f32IntegPartK_1Q_Out'], 'Position', pos, 'Orientation', orient);
      | 
      |     pos = get_param([gcb '/f16InK_1Q_Out'], 'Position');
      |     orient = get_param([gcb '/f16InK_1Q_Out'], 'Orientation');
      |     delete_block([gcb '/f16InK_1Q_Out']);
      |     add_block('built-in/Outport', [gcb '/f16InK_1Q_Out'], 'Position', pos, 'Orientation', orient);
      | 
      |     pos = get_param([gcb '/f32IntegPartK_1FW_Out'], 'Position');
      |     orient = get_param([gcb '/f32IntegPartK_1FW_Out'], 'Orientation');
      |     delete_block([gcb '/f32IntegPartK_1FW_Out']);
      |     add_block('built-in/Outport', [gcb '/f32IntegPartK_1FW_Out'], 'Position', pos, 'Orientation', orient);
      | 
      |     pos = get_param([gcb '/f16InK_1FW_Out'], 'Position');
      |     orient = get_param([gcb '/f16InK_1FW_Out'], 'Orientation');
      |     delete_block([gcb '/f16InK_1FW_Out']);
      |     add_block('built-in/Outport', [gcb '/f16InK_1FW_Out'], 'Position', pos, 'Orientation', orient);
      | 
      | 
      |     pmask=Simulink.Mask.get(gcb);
      |     pctrl=pmask.getParameter('SampleTime');
      |     pctrl.set('TypeOptions',{'f16VelocityReq/SampleTime','f16VelocityFbck/SampleTime','f16IQFbck/SampleTime','f16UQReq/SampleTime','f16UQLim/SampleTime','f16FilterMAWOut_preset/SampleTime','f16FilterMAFWOut_preset/SampleTime','f16ControllerPIpAWQOut_preset/SampleTime','f16ControllerPIpAWFWOut_preset/SampleTime','f32RampOut_preset/SampleTime','u16NSamplesW/SampleTime','u16NSamplesFW/SampleTime','f16PropGainQ/SampleTime','f16IntegGainQ/SampleTime','s16PropGainShiftQ/SampleTime','s16IntegGainShiftQ/SampleTime','f16LowerLimitQ/SampleTime','f16UpperLimitQ/SampleTime','f16PropGainFW/SampleTime','f16IntegGainFW/SampleTime','s16PropGainShiftFW/SampleTime','s16IntegGainShiftFW/SampleTime','f16LowerLimitFW/SampleTime','f16UpperLimitFW/SampleTime','f32RampUp/SampleTime','f32RampDown/SampleTime','f16IQReqK_1/SampleTime','f32AccW/SampleTime','f32AccFW/SampleTime','f32IntegPartK_1Q/SampleTime','f16InK_1Q/SampleTime','f32IntegPartK_1FW/SampleTime','f16InK_1FW/SampleTime','f32State/SampleTime'});
      | 
      |     if (showDebugOutputs == 2) && (strcmp(get_param([gcb '/f16WReqFilt'], 'BlockType'), 'Terminator'))
      |       pos = get_param([gcb '/f16WReqFilt'], 'Position');
      |       orient = get_param([gcb '/f16WReqFilt'], 'Orientation');
      |       delete_block([gcb '/f16WReqFilt']);
      |       add_block('built-in/Outport', [gcb '/f16WReqFilt'], 'Position', pos, 'Orientation', orient);
      | 
      |       pos = get_param([gcb '/f16WErr'], 'Position');
      |       orient = get_param([gcb '/f16WErr'], 'Orientation');
      |       delete_block([gcb '/f16WErr']);
      |       add_block('built-in/Outport', [gcb '/f16WErr'], 'Position', pos, 'Orientation', orient);
      | 
      |       pos = get_param([gcb '/f16IDQReqAmp'], 'Position');
      |       orient = get_param([gcb '/f16IDQReqAmp'], 'Orientation');
      |       delete_block([gcb '/f16IDQReqAmp']);
      |       add_block('built-in/Outport', [gcb '/f16IDQReqAmp'], 'Position', pos, 'Orientation', orient);
      | 
      |       pos = get_param([gcb '/f16WFbckFilt'], 'Position');
      |       orient = get_param([gcb '/f16WFbckFilt'], 'Orientation');
      |       delete_block([gcb '/f16WFbckFilt']);
      |       add_block('built-in/Outport', [gcb '/f16WFbckFilt'], 'Position', pos, 'Orientation', orient);
      | 
      |       pos = get_param([gcb '/f16IQErrSign'], 'Position');
      |       orient = get_param([gcb '/f16IQErrSign'], 'Orientation');
      |       delete_block([gcb '/f16IQErrSign']);
      |       add_block('built-in/Outport', [gcb '/f16IQErrSign'], 'Position', pos, 'Orientation', orient);
      | 
      |       pos = get_param([gcb '/f16IQErr'], 'Position');
      |       orient = get_param([gcb '/f16IQErr'], 'Orientation');
      |       delete_block([gcb '/f16IQErr']);
      |       add_block('built-in/Outport', [gcb '/f16IQErr'], 'Position', pos, 'Orientation', orient);
      | 
      |       pos = get_param([gcb '/f16FWErr'], 'Position');
      |       orient = get_param([gcb '/f16FWErr'], 'Orientation');
      |       delete_block([gcb '/f16FWErr']);
      |       add_block('built-in/Outport', [gcb '/f16FWErr'], 'Position', pos, 'Orientation', orient);
      | 
      |       pos = get_param([gcb '/f16UQErr'], 'Position');
      |       orient = get_param([gcb '/f16UQErr'], 'Orientation');
      |       delete_block([gcb '/f16UQErr']);
      |       add_block('built-in/Outport', [gcb '/f16UQErr'], 'Position', pos, 'Orientation', orient);
      | 
      |       pos = get_param([gcb '/f16FWErrFilt'], 'Position');
      |       orient = get_param([gcb '/f16FWErrFilt'], 'Orientation');
      |       delete_block([gcb '/f16FWErrFilt']);
      |       add_block('built-in/Outport', [gcb '/f16FWErrFilt'], 'Position', pos, 'Orientation', orient);
      | 
      |       pos = get_param([gcb '/f16FWAngle'], 'Position');
      |       orient = get_param([gcb '/f16FWAngle'], 'Orientation');
      |       delete_block([gcb '/f16FWAngle']);
      |       add_block('built-in/Outport', [gcb '/f16FWAngle'], 'Position', pos, 'Orientation', orient);
      | 
      |       pos = get_param([gcb '/f16FWSin'], 'Position');
      |       orient = get_param([gcb '/f16FWSin'], 'Orientation');
      |       delete_block([gcb '/f16FWSin']);
      |       add_block('built-in/Outport', [gcb '/f16FWSin'], 'Position', pos, 'Orientation', orient);
      | 
      |       pos = get_param([gcb '/f16FWCos'], 'Position');
      |       orient = get_param([gcb '/f16FWCos'], 'Orientation');
      |       delete_block([gcb '/f16FWCos']);
      |       add_block('built-in/Outport', [gcb '/f16FWCos'], 'Position', pos, 'Orientation', orient);
      | 
      |     end
      | 
      |     set_param([gcb '/f16VelocityReq'], 'Port', '1');
      |     set_param([gcb '/f16VelocityFbck'], 'Port', '2');
      |     set_param([gcb '/f16IQFbck'], 'Port', '3');
      |     set_param([gcb '/f16UQReq'], 'Port', '4');
      |     set_param([gcb '/f16UQLim'], 'Port', '5');
      |     set_param([gcb '/f16FilterMAWOut_preset'], 'Port', '6');
      |     set_param([gcb '/f16FilterMAFWOut_preset'], 'Port', '7');
      |     set_param([gcb '/f16ControllerPIpAWQOut_preset'], 'Port', '8');
      |     set_param([gcb '/f16ControllerPIpAWFWOut_preset'], 'Port', '9');
      |     set_param([gcb '/f32RampOut_preset'], 'Port', '10');
      |     set_param([gcb '/u16NSamplesW'], 'Port', '11');
      |     set_param([gcb '/u16NSamplesFW'], 'Port', '12');
      |     set_param([gcb '/f16PropGainQ'], 'Port', '13');
      |     set_param([gcb '/f16IntegGainQ'], 'Port', '14');
      |     set_param([gcb '/s16PropGainShiftQ'], 'Port', '15');
      |     set_param([gcb '/s16IntegGainShiftQ'], 'Port', '16');
      |     set_param([gcb '/f16LowerLimitQ'], 'Port', '17');
      |     set_param([gcb '/f16UpperLimitQ'], 'Port', '18');
      |     set_param([gcb '/f16PropGainFW'], 'Port', '19');
      |     set_param([gcb '/f16IntegGainFW'], 'Port', '20');
      |     set_param([gcb '/s16PropGainShiftFW'], 'Port', '21');
      |     set_param([gcb '/s16IntegGainShiftFW'], 'Port', '22');
      |     set_param([gcb '/f16LowerLimitFW'], 'Port', '23');
      |     set_param([gcb '/f16UpperLimitFW'], 'Port', '24');
      |     set_param([gcb '/f32RampUp'], 'Port', '25');
      |     set_param([gcb '/f32RampDown'], 'Port', '26');
      |     set_param([gcb '/f16IQReqK_1'], 'Port', '27');
      |     set_param([gcb '/f32AccW'], 'Port', '28');
      |     set_param([gcb '/f32AccFW'], 'Port', '29');
      |     set_param([gcb '/f32IntegPartK_1Q'], 'Port', '30');
      |     set_param([gcb '/f16InK_1Q'], 'Port', '31');
      |     set_param([gcb '/f32IntegPartK_1FW'], 'Port', '32');
      |     set_param([gcb '/f16InK_1FW'], 'Port', '33');
      |     set_param([gcb '/f32State'], 'Port', '34');
      | 
      |     if (showDebugOutputs == 2)
      |       tmpOutCnt=0;
      |       tmpOutCnt=tmpOutCnt+1;
      |       set_param([gcb '/pIDQReq'], 'Port', num2str(tmpOutCnt));
      |       tmpOutCnt=tmpOutCnt+1;
      |       set_param([gcb '/u16LimitFlagQ'], 'Port', num2str(tmpOutCnt));
      |       tmpOutCnt=tmpOutCnt+1;
      |       set_param([gcb '/u16LimitFlagFW'], 'Port', num2str(tmpOutCnt));
      |       tmpOutCnt=tmpOutCnt+1;
      |       set_param([gcb '/f16WReqFilt'], 'Port', num2str(tmpOutCnt));
      |       tmpOutCnt=tmpOutCnt+1;
      |       set_param([gcb '/f16WErr'], 'Port', num2str(tmpOutCnt));
      |       tmpOutCnt=tmpOutCnt+1;
      |       set_param([gcb '/f16IDQReqAmp'], 'Port', num2str(tmpOutCnt));
      |       tmpOutCnt=tmpOutCnt+1;
      |       set_param([gcb '/f16WFbckFilt'], 'Port', num2str(tmpOutCnt));
      |       tmpOutCnt=tmpOutCnt+1;
      |       set_param([gcb '/f16IQErrSign'], 'Port', num2str(tmpOutCnt));
      |       tmpOutCnt=tmpOutCnt+1;
      |       set_param([gcb '/f16IQErr'], 'Port', num2str(tmpOutCnt));
      |       tmpOutCnt=tmpOutCnt+1;
      |       set_param([gcb '/f16FWErr'], 'Port', num2str(tmpOutCnt));
      |       tmpOutCnt=tmpOutCnt+1;
      |       set_param([gcb '/f16UQErr'], 'Port', num2str(tmpOutCnt));
      |       tmpOutCnt=tmpOutCnt+1;
      |       set_param([gcb '/f16FWErrFilt'], 'Port', num2str(tmpOutCnt));
      |       tmpOutCnt=tmpOutCnt+1;
      |       set_param([gcb '/f16FWAngle'], 'Port', num2str(tmpOutCnt));
      |       tmpOutCnt=tmpOutCnt+1;
      |       set_param([gcb '/f16FWSin'], 'Port', num2str(tmpOutCnt));
      |       tmpOutCnt=tmpOutCnt+1;
      |       set_param([gcb '/f16FWCos'], 'Port', num2str(tmpOutCnt));
      |       tmpOutCnt=tmpOutCnt+1;
      |       set_param([gcb '/f32AccW_Out'], 'Port', num2str(tmpOutCnt));
      |       tmpOutCnt=tmpOutCnt+1;
      |       set_param([gcb '/f32AccFW_Out'], 'Port', num2str(tmpOutCnt));
      |       tmpOutCnt=tmpOutCnt+1;
      |       set_param([gcb '/f32IntegPartK_1Q_Out'], 'Port', num2str(tmpOutCnt));
      |       tmpOutCnt=tmpOutCnt+1;
      |       set_param([gcb '/f16InK_1Q_Out'], 'Port', num2str(tmpOutCnt));
      |       tmpOutCnt=tmpOutCnt+1;
      |       set_param([gcb '/f32IntegPartK_1FW_Out'], 'Port', num2str(tmpOutCnt));
      |       tmpOutCnt=tmpOutCnt+1;
      |       set_param([gcb '/f16InK_1FW_Out'], 'Port', num2str(tmpOutCnt));
      |       if strcmp(get_param([gcb '/f32State_Out'], 'BlockType'), 'Outport')
      |         tmpOutCnt=tmpOutCnt+1;
      |         set_param([gcb '/f32State_Out'], 'Port', num2str(tmpOutCnt));
      |       end
      |     else
      |       tmpOutCnt=0;
      |       tmpOutCnt=tmpOutCnt+1;
      |       set_param([gcb '/pIDQReq'], 'Port', num2str(tmpOutCnt));
      |       tmpOutCnt=tmpOutCnt+1;
      |       set_param([gcb '/u16LimitFlagQ'], 'Port', num2str(tmpOutCnt));
      |       tmpOutCnt=tmpOutCnt+1;
      |       set_param([gcb '/u16LimitFlagFW'], 'Port', num2str(tmpOutCnt));
      |       tmpOutCnt=tmpOutCnt+1;
      |       set_param([gcb '/f32AccW_Out'], 'Port', num2str(tmpOutCnt));
      |       tmpOutCnt=tmpOutCnt+1;
      |       set_param([gcb '/f32AccFW_Out'], 'Port', num2str(tmpOutCnt));
      |       tmpOutCnt=tmpOutCnt+1;
      |       set_param([gcb '/f32IntegPartK_1Q_Out'], 'Port', num2str(tmpOutCnt));
      |       tmpOutCnt=tmpOutCnt+1;
      |       set_param([gcb '/f16InK_1Q_Out'], 'Port', num2str(tmpOutCnt));
      |       tmpOutCnt=tmpOutCnt+1;
      |       set_param([gcb '/f32IntegPartK_1FW_Out'], 'Port', num2str(tmpOutCnt));
      |       tmpOutCnt=tmpOutCnt+1;
      |       set_param([gcb '/f16InK_1FW_Out'], 'Port', num2str(tmpOutCnt));
      |       if strcmp(get_param([gcb '/f32State_Out'], 'BlockType'), 'Outport')
      |         tmpOutCnt=tmpOutCnt+1;
      |         set_param([gcb '/f32State_Out'], 'Port', num2str(tmpOutCnt));
      |       end
      |     end
      | 
      |     set_param(gcb,'MaskEnables',{'on','on','on','on','on','off','off','off','off','off','off','off','off','off','off','off','off','off','off','off','off','off','off','off','off','off','off','off','off','off','off','off','off','off','off'});
      | 
      |     if (posblk(4) - posblk(2)) < 875
      |       height = 875;
      |       set_param(gcb,'Position',[posblk(1), posblk(2), posblk(3), posblk(2)+height])
      |     end
      |   else
      |     if (showDebugOutputs == 2) && (strcmp(get_param([gcb '/f16WReqFilt'], 'BlockType'), 'Terminator'))
      |       % shown debugging outputs
      |       pos = get_param([gcb '/f16WReqFilt'], 'Position');
      |       orient = get_param([gcb '/f16WReqFilt'], 'Orientation');
      |       delete_block([gcb '/f16WReqFilt']);
      |       add_block('built-in/Outport', [gcb '/f16WReqFilt'], 'Position', pos, 'Orientation', orient);
      | 
      |       pos = get_param([gcb '/f16WErr'], 'Position');
      |       orient = get_param([gcb '/f16WErr'], 'Orientation');
      |       delete_block([gcb '/f16WErr']);
      |       add_block('built-in/Outport', [gcb '/f16WErr'], 'Position', pos, 'Orientation', orient);
      | 
      |       pos = get_param([gcb '/f16IDQReqAmp'], 'Position');
      |       orient = get_param([gcb '/f16IDQReqAmp'], 'Orientation');
      |       delete_block([gcb '/f16IDQReqAmp']);
      |       add_block('built-in/Outport', [gcb '/f16IDQReqAmp'], 'Position', pos, 'Orientation', orient);
      | 
      |       pos = get_param([gcb '/f16WFbckFilt'], 'Position');
      |       orient = get_param([gcb '/f16WFbckFilt'], 'Orientation');
      |       delete_block([gcb '/f16WFbckFilt']);
      |       add_block('built-in/Outport', [gcb '/f16WFbckFilt'], 'Position', pos, 'Orientation', orient);
      | 
      |       pos = get_param([gcb '/f16IQErrSign'], 'Position');
      |       orient = get_param([gcb '/f16IQErrSign'], 'Orientation');
      |       delete_block([gcb '/f16IQErrSign']);
      |       add_block('built-in/Outport', [gcb '/f16IQErrSign'], 'Position', pos, 'Orientation', orient);
      | 
      |       pos = get_param([gcb '/f16IQErr'], 'Position');
      |       orient = get_param([gcb '/f16IQErr'], 'Orientation');
      |       delete_block([gcb '/f16IQErr']);
      |       add_block('built-in/Outport', [gcb '/f16IQErr'], 'Position', pos, 'Orientation', orient);
      | 
      |       pos = get_param([gcb '/f16FWErr'], 'Position');
      |       orient = get_param([gcb '/f16FWErr'], 'Orientation');
      |       delete_block([gcb '/f16FWErr']);
      |       add_block('built-in/Outport', [gcb '/f16FWErr'], 'Position', pos, 'Orientation', orient);
      | 
      |       pos = get_param([gcb '/f16UQErr'], 'Position');
      |       orient = get_param([gcb '/f16UQErr'], 'Orientation');
      |       delete_block([gcb '/f16UQErr']);
      |       add_block('built-in/Outport', [gcb '/f16UQErr'], 'Position', pos, 'Orientation', orient);
      | 
      |       pos = get_param([gcb '/f16FWErrFilt'], 'Position');
      |       orient = get_param([gcb '/f16FWErrFilt'], 'Orientation');
      |       delete_block([gcb '/f16FWErrFilt']);
      |       add_block('built-in/Outport', [gcb '/f16FWErrFilt'], 'Position', pos, 'Orientation', orient);
      | 
      |       pos = get_param([gcb '/f16FWAngle'], 'Position');
      |       orient = get_param([gcb '/f16FWAngle'], 'Orientation');
      |       delete_block([gcb '/f16FWAngle']);
      |       add_block('built-in/Outport', [gcb '/f16FWAngle'], 'Position', pos, 'Orientation', orient);
      | 
      |       pos = get_param([gcb '/f16FWSin'], 'Position');
      |       orient = get_param([gcb '/f16FWSin'], 'Orientation');
      |       delete_block([gcb '/f16FWSin']);
      |       add_block('built-in/Outport', [gcb '/f16FWSin'], 'Position', pos, 'Orientation', orient);
      | 
      |       pos = get_param([gcb '/f16FWCos'], 'Position');
      |       orient = get_param([gcb '/f16FWCos'], 'Orientation');
      |       delete_block([gcb '/f16FWCos']);
      |       add_block('built-in/Outport', [gcb '/f16FWCos'], 'Position', pos, 'Orientation', orient);
      | 
      |       tmpOutCnt=0;
      |       tmpOutCnt=tmpOutCnt+1;
      |       set_param([gcb '/pIDQReq'], 'Port', num2str(tmpOutCnt));
      |       tmpOutCnt=tmpOutCnt+1;
      |       set_param([gcb '/u16LimitFlagQ'], 'Port', num2str(tmpOutCnt));
      |       tmpOutCnt=tmpOutCnt+1;
      |       set_param([gcb '/u16LimitFlagFW'], 'Port', num2str(tmpOutCnt));
      |       tmpOutCnt=tmpOutCnt+1;
      |       set_param([gcb '/f16WReqFilt'], 'Port', num2str(tmpOutCnt));
      |       tmpOutCnt=tmpOutCnt+1;
      |       set_param([gcb '/f16WErr'], 'Port', num2str(tmpOutCnt));
      |       tmpOutCnt=tmpOutCnt+1;
      |       set_param([gcb '/f16IDQReqAmp'], 'Port', num2str(tmpOutCnt));
      |       tmpOutCnt=tmpOutCnt+1;
      |       set_param([gcb '/f16WFbckFilt'], 'Port', num2str(tmpOutCnt));
      |       tmpOutCnt=tmpOutCnt+1;
      |       set_param([gcb '/f16IQErrSign'], 'Port', num2str(tmpOutCnt));
      |       tmpOutCnt=tmpOutCnt+1;
      |       set_param([gcb '/f16IQErr'], 'Port', num2str(tmpOutCnt));
      |       tmpOutCnt=tmpOutCnt+1;
      |       set_param([gcb '/f16FWErr'], 'Port', num2str(tmpOutCnt));
      |       tmpOutCnt=tmpOutCnt+1;
      |       set_param([gcb '/f16UQErr'], 'Port', num2str(tmpOutCnt));
      |       tmpOutCnt=tmpOutCnt+1;
      |       set_param([gcb '/f16FWErrFilt'], 'Port', num2str(tmpOutCnt));
      |       tmpOutCnt=tmpOutCnt+1;
      |       set_param([gcb '/f16FWAngle'], 'Port', num2str(tmpOutCnt));
      |       tmpOutCnt=tmpOutCnt+1;
      |       set_param([gcb '/f16FWSin'], 'Port', num2str(tmpOutCnt));
      |       tmpOutCnt=tmpOutCnt+1;
      |       set_param([gcb '/f16FWCos'], 'Port', num2str(tmpOutCnt));
      |       tmpOutCnt=tmpOutCnt+1;
      |       set_param([gcb '/f32AccW_Out'], 'Port', num2str(tmpOutCnt));
      |       tmpOutCnt=tmpOutCnt+1;
      |       set_param([gcb '/f32AccFW_Out'], 'Port', num2str(tmpOutCnt));
      |       tmpOutCnt=tmpOutCnt+1;
      |       set_param([gcb '/f32IntegPartK_1Q_Out'], 'Port', num2str(tmpOutCnt));
      |       tmpOutCnt=tmpOutCnt+1;
      |       set_param([gcb '/f16InK_1Q_Out'], 'Port', num2str(tmpOutCnt));
      |       tmpOutCnt=tmpOutCnt+1;
      |       set_param([gcb '/f32IntegPartK_1FW_Out'], 'Port', num2str(tmpOutCnt));
      |       tmpOutCnt=tmpOutCnt+1;
      |       set_param([gcb '/f16InK_1FW_Out'], 'Port', num2str(tmpOutCnt));
      |       if strcmp(get_param([gcb '/f32State_Out'], 'BlockType'), 'Outport')
      |         tmpOutCnt=tmpOutCnt+1;
      |         set_param([gcb '/f32State_Out'], 'Port', num2str(tmpOutCnt));
      |       end
      |     elseif (showDebugOutputs == 1) && (strcmp(get_param([gcb '/f16WReqFilt'], 'BlockType'), 'Outport'))
      |       % hidden debugging outputs
      |       pos = get_param([gcb '/f16WReqFilt'], 'Position');
      |       orient = get_param([gcb '/f16WReqFilt'], 'Orientation');
      |       delete_block([gcb '/f16WReqFilt']);
      |       add_block('built-in/Terminator', [gcb '/f16WReqFilt'], 'Position', pos, 'Orientation', orient);
      | 
      |       pos = get_param([gcb '/f16WErr'], 'Position');
      |       orient = get_param([gcb '/f16WErr'], 'Orientation');
      |       delete_block([gcb '/f16WErr']);
      |       add_block('built-in/Terminator', [gcb '/f16WErr'], 'Position', pos, 'Orientation', orient);
      | 
      |       pos = get_param([gcb '/f16IDQReqAmp'], 'Position');
      |       orient = get_param([gcb '/f16IDQReqAmp'], 'Orientation');
      |       delete_block([gcb '/f16IDQReqAmp']);
      |       add_block('built-in/Terminator', [gcb '/f16IDQReqAmp'], 'Position', pos, 'Orientation', orient);
      | 
      |       pos = get_param([gcb '/f16WFbckFilt'], 'Position');
      |       orient = get_param([gcb '/f16WFbckFilt'], 'Orientation');
      |       delete_block([gcb '/f16WFbckFilt']);
      |       add_block('built-in/Terminator', [gcb '/f16WFbckFilt'], 'Position', pos, 'Orientation', orient);
      | 
      |       pos = get_param([gcb '/f16IQErrSign'], 'Position');
      |       orient = get_param([gcb '/f16IQErrSign'], 'Orientation');
      |       delete_block([gcb '/f16IQErrSign']);
      |       add_block('built-in/Terminator', [gcb '/f16IQErrSign'], 'Position', pos, 'Orientation', orient);
      | 
      |       pos = get_param([gcb '/f16IQErr'], 'Position');
      |       orient = get_param([gcb '/f16IQErr'], 'Orientation');
      |       delete_block([gcb '/f16IQErr']);
      |       add_block('built-in/Terminator', [gcb '/f16IQErr'], 'Position', pos, 'Orientation', orient);
      | 
      |       pos = get_param([gcb '/f16FWErr'], 'Position');
      |       orient = get_param([gcb '/f16FWErr'], 'Orientation');
      |       delete_block([gcb '/f16FWErr']);
      |       add_block('built-in/Terminator', [gcb '/f16FWErr'], 'Position', pos, 'Orientation', orient);
      | 
      |       pos = get_param([gcb '/f16UQErr'], 'Position');
      |       orient = get_param([gcb '/f16UQErr'], 'Orientation');
      |       delete_block([gcb '/f16UQErr']);
      |       add_block('built-in/Terminator', [gcb '/f16UQErr'], 'Position', pos, 'Orientation', orient);
      | 
      |       pos = get_param([gcb '/f16FWErrFilt'], 'Position');
      |       orient = get_param([gcb '/f16FWErrFilt'], 'Orientation');
      |       delete_block([gcb '/f16FWErrFilt']);
      |       add_block('built-in/Terminator', [gcb '/f16FWErrFilt'], 'Position', pos, 'Orientation', orient);
      | 
      |       pos = get_param([gcb '/f16FWAngle'], 'Position');
      |       orient = get_param([gcb '/f16FWAngle'], 'Orientation');
      |       delete_block([gcb '/f16FWAngle']);
      |       add_block('built-in/Terminator', [gcb '/f16FWAngle'], 'Position', pos, 'Orientation', orient);
      | 
      |       pos = get_param([gcb '/f16FWSin'], 'Position');
      |       orient = get_param([gcb '/f16FWSin'], 'Orientation');
      |       delete_block([gcb '/f16FWSin']);
      |       add_block('built-in/Terminator', [gcb '/f16FWSin'], 'Position', pos, 'Orientation', orient);
      | 
      |       pos = get_param([gcb '/f16FWCos'], 'Position');
      |       orient = get_param([gcb '/f16FWCos'], 'Orientation');
      |       delete_block([gcb '/f16FWCos']);
      |       add_block('built-in/Terminator', [gcb '/f16FWCos'], 'Position', pos, 'Orientation', orient);
      | 
      |       tmpOutCnt=0;
      |       tmpOutCnt=tmpOutCnt+1;
      |       set_param([gcb '/pIDQReq'], 'Port', num2str(tmpOutCnt));
      |       tmpOutCnt=tmpOutCnt+1;
      |       set_param([gcb '/u16LimitFlagQ'], 'Port', num2str(tmpOutCnt));
      |       tmpOutCnt=tmpOutCnt+1;
      |       set_param([gcb '/u16LimitFlagFW'], 'Port', num2str(tmpOutCnt));
      |       tmpOutCnt=tmpOutCnt+1;
      |       set_param([gcb '/f32AccW_Out'], 'Port', num2str(tmpOutCnt));
      |       tmpOutCnt=tmpOutCnt+1;
      |       set_param([gcb '/f32AccFW_Out'], 'Port', num2str(tmpOutCnt));
      |       tmpOutCnt=tmpOutCnt+1;
      |       set_param([gcb '/f32IntegPartK_1Q_Out'], 'Port', num2str(tmpOutCnt));
      |       tmpOutCnt=tmpOutCnt+1;
      |       set_param([gcb '/f16InK_1Q_Out'], 'Port', num2str(tmpOutCnt));
      |       tmpOutCnt=tmpOutCnt+1;
      |       set_param([gcb '/f32IntegPartK_1FW_Out'], 'Port', num2str(tmpOutCnt));
      |       tmpOutCnt=tmpOutCnt+1;
      |       set_param([gcb '/f16InK_1FW_Out'], 'Port', num2str(tmpOutCnt));
      |       if strcmp(get_param([gcb '/f32State_Out'], 'BlockType'), 'Outport')
      |         tmpOutCnt=tmpOutCnt+1;
      |         set_param([gcb '/f32State_Out'], 'Port', num2str(tmpOutCnt));
      |       end
      |     end
      |   end
      | end
      | if strcmp(get_param(gcb,'f32State_Out_showOutput'),'on')
      |   if strcmp(get_param([gcb '/f32State_Out'], 'BlockType'), 'Terminator')
      |     pos = get_param([gcb '/f32State_Out'], 'Position');
      |     orient = get_param([gcb '/f32State_Out'], 'Orientation');
      |     delete_block([gcb '/f32State_Out']);
      |     add_block('built-in/Outport', [gcb '/f32State_Out'], 'Position', pos, 'Orientation', orient);
      |     outputsChanged = 1;
      |   end
      | else
      |   if strcmp(get_param([gcb '/f32State_Out'], 'BlockType'), 'Outport')
      |     pos = get_param([gcb '/f32State_Out'], 'Position');
      |     orient = get_param([gcb '/f32State_Out'], 'Orientation');
      |     delete_block([gcb '/f32State_Out']);
      |     add_block('built-in/Terminator', [gcb '/f32State_Out'], 'Position', pos, 'Orientation', orient);
      |     outputsChanged = 1;
      |   end
      | end
      | if outputsChanged == 1;
      |   tmpOutCnt = 0;
      |   if strcmp(get_param([gcb '/pIDQReq'], 'BlockType'), 'Outport')
      |     tmpOutCnt = tmpOutCnt + 1;
      |     set_param([gcb '/pIDQReq'], 'Port', num2str(tmpOutCnt));
      |   end
      |   if strcmp(get_param([gcb '/u16LimitFlagQ'], 'BlockType'), 'Outport')
      |     tmpOutCnt = tmpOutCnt + 1;
      |     set_param([gcb '/u16LimitFlagQ'], 'Port', num2str(tmpOutCnt));
      |   end
      |   if strcmp(get_param([gcb '/u16LimitFlagFW'], 'BlockType'), 'Outport')
      |     tmpOutCnt = tmpOutCnt + 1;
      |     set_param([gcb '/u16LimitFlagFW'], 'Port', num2str(tmpOutCnt));
      |   end
      |   if strcmp(get_param([gcb '/f16WReqFilt'], 'BlockType'), 'Outport')
      |     tmpOutCnt = tmpOutCnt + 1;
      |     set_param([gcb '/f16WReqFilt'], 'Port', num2str(tmpOutCnt));
      |   end
      |   if strcmp(get_param([gcb '/f16WErr'], 'BlockType'), 'Outport')
      |     tmpOutCnt = tmpOutCnt + 1;
      |     set_param([gcb '/f16WErr'], 'Port', num2str(tmpOutCnt));
      |   end
      |   if strcmp(get_param([gcb '/f16IDQReqAmp'], 'BlockType'), 'Outport')
      |     tmpOutCnt = tmpOutCnt + 1;
      |     set_param([gcb '/f16IDQReqAmp'], 'Port', num2str(tmpOutCnt));
      |   end
      |   if strcmp(get_param([gcb '/f16WFbckFilt'], 'BlockType'), 'Outport')
      |     tmpOutCnt = tmpOutCnt + 1;
      |     set_param([gcb '/f16WFbckFilt'], 'Port', num2str(tmpOutCnt));
      |   end
      |   if strcmp(get_param([gcb '/f16IQErrSign'], 'BlockType'), 'Outport')
      |     tmpOutCnt = tmpOutCnt + 1;
      |     set_param([gcb '/f16IQErrSign'], 'Port', num2str(tmpOutCnt));
      |   end
      |   if strcmp(get_param([gcb '/f16IQErr'], 'BlockType'), 'Outport')
      |     tmpOutCnt = tmpOutCnt + 1;
      |     set_param([gcb '/f16IQErr'], 'Port', num2str(tmpOutCnt));
      |   end
      |   if strcmp(get_param([gcb '/f16FWErr'], 'BlockType'), 'Outport')
      |     tmpOutCnt = tmpOutCnt + 1;
      |     set_param([gcb '/f16FWErr'], 'Port', num2str(tmpOutCnt));
      |   end
      |   if strcmp(get_param([gcb '/f16UQErr'], 'BlockType'), 'Outport')
      |     tmpOutCnt = tmpOutCnt + 1;
      |     set_param([gcb '/f16UQErr'], 'Port', num2str(tmpOutCnt));
      |   end
      |   if strcmp(get_param([gcb '/f16FWErrFilt'], 'BlockType'), 'Outport')
      |     tmpOutCnt = tmpOutCnt + 1;
      |     set_param([gcb '/f16FWErrFilt'], 'Port', num2str(tmpOutCnt));
      |   end
      |   if strcmp(get_param([gcb '/f16FWAngle'], 'BlockType'), 'Outport')
      |     tmpOutCnt = tmpOutCnt + 1;
      |     set_param([gcb '/f16FWAngle'], 'Port', num2str(tmpOutCnt));
      |   end
      |   if strcmp(get_param([gcb '/f16FWSin'], 'BlockType'), 'Outport')
      |     tmpOutCnt = tmpOutCnt + 1;
      |     set_param([gcb '/f16FWSin'], 'Port', num2str(tmpOutCnt));
      |   end
      |   if strcmp(get_param([gcb '/f16FWCos'], 'BlockType'), 'Outport')
      |     tmpOutCnt = tmpOutCnt + 1;
      |     set_param([gcb '/f16FWCos'], 'Port', num2str(tmpOutCnt));
      |   end
      |   if strcmp(get_param([gcb '/f32AccW_Out'], 'BlockType'), 'Outport')
      |     tmpOutCnt = tmpOutCnt + 1;
      |     set_param([gcb '/f32AccW_Out'], 'Port', num2str(tmpOutCnt));
      |   end
      |   if strcmp(get_param([gcb '/f32AccFW_Out'], 'BlockType'), 'Outport')
      |     tmpOutCnt = tmpOutCnt + 1;
      |     set_param([gcb '/f32AccFW_Out'], 'Port', num2str(tmpOutCnt));
      |   end
      |   if strcmp(get_param([gcb '/f32IntegPartK_1Q_Out'], 'BlockType'), 'Outport')
      |     tmpOutCnt = tmpOutCnt + 1;
      |     set_param([gcb '/f32IntegPartK_1Q_Out'], 'Port', num2str(tmpOutCnt));
      |   end
      |   if strcmp(get_param([gcb '/f16InK_1Q_Out'], 'BlockType'), 'Outport')
      |     tmpOutCnt = tmpOutCnt + 1;
      |     set_param([gcb '/f16InK_1Q_Out'], 'Port', num2str(tmpOutCnt));
      |   end
      |   if strcmp(get_param([gcb '/f32IntegPartK_1FW_Out'], 'BlockType'), 'Outport')
      |     tmpOutCnt = tmpOutCnt + 1;
      |     set_param([gcb '/f32IntegPartK_1FW_Out'], 'Port', num2str(tmpOutCnt));
      |   end
      |   if strcmp(get_param([gcb '/f16InK_1FW_Out'], 'BlockType'), 'Outport')
      |     tmpOutCnt = tmpOutCnt + 1;
      |     set_param([gcb '/f16InK_1FW_Out'], 'Port', num2str(tmpOutCnt));
      |   end
      |   if strcmp(get_param([gcb '/f32State_Out'], 'BlockType'), 'Outport')
      |     tmpOutCnt = tmpOutCnt + 1;
      |     set_param([gcb '/f32State_Out'], 'Port', num2str(tmpOutCnt));
      |   end
      | end
      settings: RTWSystemCode=Inline
      mask Help: web([fileparts(which('ammclib_bam_S32K3xx.slx')) '/../doc/S32K3XXMCLUG.pdf'], '-browser')
      mask TypeOptions showStates: Hide (faster execution) | Show (allows debugging; connect feedback loops manually)
      mask Callback showStates:
      | maskStr=get_param(gcb,'showStates');
      | if strcmp(maskStr,'Hide (faster execution)')
      |   autoCalcEn=get_param(gcb,'autoCalcEn');
      |   if strcmp(autoCalcEn,'on')
      |     set_param(gcb,'MaskEnables',{'on','on','off','on','on','on','on','on','on','on','on','on','on','on','on','on','on','on','on','on','on','on','on','on','on','on','on','on','on','on','on','on','on','on','off'});
      |   else
      |     set_param(gcb,'MaskEnables',{'on','on','off','on','on','off','off','off','off','off','off','off','off','off','off','off','off','on','on','on','on','on','on','on','on','on','on','on','on','on','on','on','on','on','off'});
      |   end
      | else
      |   set_param(gcb,'MaskEnables',{'on','on','on','on','on','off','off','off','off','off','off','off','off','off','off','off','off','off','off','off','off','off','off','off','off','off','off','off','off','off','off','off','off','off','off'});
      | end
      mask TypeOptions resetStatesEnable: Pre-set according to the first set of inputs after reset | Clear to zero
      mask TypeOptions showDebugOutputs: Hide | Show
      mask TypeOptions SampleTime: f16VelocityReq/SampleTime | f16VelocityFbck/SampleTime | f16IQFbck/SampleTime | f16UQReq/SampleTime | f16UQLim/SampleTime | f16FilterMAWOut_preset/SampleTime | f16FilterMAFWOut_preset/SampleTime | f16ControllerPIpAWQOut_preset/SampleTime | f16ControllerPIpAWFWOut_preset/SampleTime | f32RampOut_preset/SampleTime
      mask Callback SampleTime:
      | p=Simulink.Mask.get(gcb);
      | hintText=p.getDialogControl('timeHint');
      | SampleTime=Simulink.data.evalinGlobal(bdroot,get_param(gcb,'SampleTime'));
      | SampleTime_1=str2double(get_param(gcb,'SampleTime_1'));
      | if (((SampleTime==-1) && (~contains(hintText.Prompt,'inherited'))) || ...
      |     ((SampleTime~=-1) && contains(hintText.Prompt,'inherited')) || ...
      |     ((SampleTime~=-1) && (SampleTime_1~=SampleTime)) || ...
      |     ((SampleTime_1~=-1) && contains(hintText.Prompt,'yet')))
      |   if ((SampleTime==-1) && (~contains(hintText.Prompt,'inherited')))
      |     set_param(gcb,'SampleTime_1',num2str(NaN));
      |     SampleTime_1=NaN;
      |   end
      |   if (SampleTime~=-1)
      |     set_param(gcb,'SampleTime_1',num2str(SampleTime));
      |     SampleTime_1=SampleTime;
      |   end
      |   autoCalcEn=get_param(gcb,'autoCalcEn');
      |   if strcmp(autoCalcEn,'on')
      |     p=Simulink.Mask.get(gcb);
      |     hintText=p.getDialogControl('timeHint');
      |     if SampleTime==-1
      |       SampleTime=SampleTime_1;
      |       if isnan(SampleTime)
      |         hintText.Prompt='Note: Implementation parameters cannot be calculated yet because the block''s inherited sample time is unknown. Simulink will update the sample time when you run the simulation.';
      |       else
      |         hintText.Prompt='Caution: Implementation parameters depend on inherited sample time. Make sure that the sample time of the block''s inputs corresponds to the sampling period in the target application.';
      |       end
      |     else
      |       hintText.Prompt='Caution: Implementation parameters depend on the sample time. Make sure that the simulation time step corresponds to the sampling period in the target application.';
      |     end
      |     u16NSamplesW_bkup=get_param(gcb,'u16NSamplesW');
      |     u16NSamplesFW_bkup=get_param(gcb,'u16NSamplesFW');
      |     f16PropGainQ_bkup=get_param(gcb,'f16PropGainQ');
      |     f16IntegGainQ_bkup=get_param(gcb,'f16IntegGainQ');
      |     s16PropGainShiftQ_bkup=get_param(gcb,'s16PropGainShiftQ');
      |     s16IntegGainShiftQ_bkup=get_param(gcb,'s16IntegGainShiftQ');
      |     f16LowerLimitQ_bkup=get_param(gcb,'f16LowerLimitQ');
      |     f16UpperLimitQ_bkup=get_param(gcb,'f16UpperLimitQ');
      |     f16PropGainFW_bkup=get_param(gcb,'f16PropGainFW');
      |     f16IntegGainFW_bkup=get_param(gcb,'f16IntegGainFW');
      |     s16PropGainShiftFW_bkup=get_param(gcb,'s16PropGainShiftFW');
      |     s16IntegGainShiftFW_bkup=get_param(gcb,'s16IntegGainShiftFW');
      |     f16LowerLimitFW_bkup=get_param(gcb,'f16LowerLimitFW');
      |     f16UpperLimitFW_bkup=get_param(gcb,'f16UpperLimitFW');
      |     f32RampUp_bkup=get_param(gcb,'f32RampUp');
      |     f32RampDown_bkup=get_param(gcb,'f32RampDown');
      |     wf0=Simulink.data.evalinGlobal(bdroot,get_param(gcb,'wf0'));
      |     wksi=Simulink.data.evalinGlobal(bdroot,get_param(gcb,'wksi'));
      |     J=Simulink.data.evalinGlobal(bdroot,get_param(gcb,'J'));
      |     Kt=Simulink.data.evalinGlobal(bdroot,get_param(gcb,'Kt'));
      |     lambdaW=Simulink.data.evalinGlobal(bdroot,get_param(gcb,'lambdaW'));
      |     lambdaFW=Simulink.data.evalinGlobal(bdroot,get_param(gcb,'lambdaFW'));
      |     Idmax=Simulink.data.evalinGlobal(bdroot,get_param(gcb,'Idmax'));
      |     ramprpm=Simulink.data.evalinGlobal(bdroot,get_param(gcb,'ramprpm'));
      |     mechspeed=Simulink.data.evalinGlobal(bdroot,get_param(gcb,'mechspeed'));
      |     polepairs=Simulink.data.evalinGlobal(bdroot,get_param(gcb,'polepairs'));
      |     uscale=Simulink.data.evalinGlobal(bdroot,get_param(gcb,'uscale'));
      |     iscale=Simulink.data.evalinGlobal(bdroot,get_param(gcb,'iscale'));
      |     if (wf0<=0)
      |       warning('Natural frequency f0 must be positive.');
      |     end
      |     if (wksi<=0)
      |       warning('Current loop attenuation must be positive.');
      |     end
      |     if (wksi>1)
      |       warning('Current loop attenuation must not exceed 1.');
      |     end
      |     if (J<=0)
      |       warning('Moment of inertia J must be positive.');
      |     end
      |     if (Kt<=0)
      |       warning('Torque constant Kt must be positive.');
      |     end
      |     if (lambdaW<0)
      |       warning('MA filter smoothing factor must be in the range 0..1.');
      |     end
      |     if (lambdaW>1)
      |       warning('MA filter smoothing factor must be in the range 0..1.');
      |     end
      |     if (lambdaFW<0)
      |       warning('MA filter smoothing factor must be in the range 0..1.');
      |     end
      |     if (lambdaFW>1)
      |       warning('MA filter smoothing factor must be in the range 0..1.');
      |     end
      |     if (mechspeed<=0)
      |       warning('Max. speed must be positive.');
      |     end
      |     if (polepairs<1)
      |       warning('Number of pole pairs must be a natural number (1, 2, 3, ...).');
      |     end
      |     if (round(polepairs)~=polepairs)
      |       warning('Number of pole pairs must be a natural number (1, 2, 3, ...).');
      |     end
      |     if (uscale<=0)
      |       warning('U_max must be positive.');
      |     end
      |     if (iscale<=0)
      |       warning('I_max must be positive.');
      |     end
      |     w0=6.283185307179586*wf0;
      |     pgain=2.0*wksi*w0*J/Kt;
      |     igain=w0*w0*J/Kt;
      |     wmax=polepairs*mechspeed*0.1047197551196598;
      |     kpf=pgain*wmax/iscale;
      |     s16PropGainShiftQ=ceil(log2(abs(kpf)));
      |     if s16PropGainShiftQ<-15
      |       s16PropGainShiftQ=-15;
      |     end
      |     if s16PropGainShiftQ>15
      |       s16PropGainShiftQ=15;
      |       warning(['Parameter s16PropGainShiftQ of ' gcb ' exceeds the fixed-point range.']);
      |     end
      |     f16PropGainQ=round(kpf*2^(-s16PropGainShiftQ)*2^15);
      |     if f16PropGainQ>2^15-1
      |       f16PropGainQ=2^15-1;
      |       warning(['Parameter f16PropGainQ of ' gcb ' exceeds the fixed-point range.']);
      |     end
      |     if f16PropGainQ<-2^15
      |       f16PropGainQ=-2^15;
      |       warning(['Parameter f16PropGainQ of ' gcb ' exceeds the fixed-point range.']);
      |     end
      |     kif=igain*SampleTime*0.5*wmax/iscale;
      |     s16IntegGainShiftQ=ceil(log2(abs(kif)));
      |     if s16IntegGainShiftQ<-15
      |       s16IntegGainShiftQ=-15;
      |     end
      |     if s16IntegGainShiftQ>15
      |       s16IntegGainShiftQ=15;
      |       warning(['Parameter s16IntegGainShiftQ of ' gcb ' exceeds the fixed-point range.']);
      |     end
      |     f16IntegGainQ=round(kif*2^(-s16IntegGainShiftQ)*2^15);
      |     if f16IntegGainQ>2^15-1
      |       f16IntegGainQ=2^15-1;
      |       warning(['Parameter f16IntegGainQ of ' gcb ' exceeds the fixed-point range.']);
      |     end
      |     if f16IntegGainQ<-2^15
      |       f16IntegGainQ=-2^15;
      |       warning(['Parameter f16IntegGainQ of ' gcb ' exceeds the fixed-point range.']);
      |     end
      |     f16LowerLimitQ=-32768;
      |     f16UpperLimitQ=32767;
      |     fwkpf=0.9*pgain*wmax/iscale;
      |     s16PropGainShiftFW=ceil(log2(abs(fwkpf)));
      |     if s16PropGainShiftFW<-15
      |       s16PropGainShiftFW=-15;
      |     end
      |     if s16PropGainShiftFW>15
      |       s16PropGainShiftFW=15;
      |       warning(['Parameter s16PropGainShiftFW of ' gcb ' exceeds the fixed-point range.']);
      |     end
      |     f16PropGainFW=round(fwkpf*2^(-s16PropGainShiftFW)*2^15);
      |     if f16PropGainFW>2^15-1
      |       f16PropGainFW=2^15-1;
      |       warning(['Parameter f16PropGainFW of ' gcb ' exceeds the fixed-point range.']);
      |     end
      |     if f16PropGainFW<-2^15
      |       f16PropGainFW=-2^15;
      |       warning(['Parameter f16PropGainFW of ' gcb ' exceeds the fixed-point range.']);
      |     end
      |     s16IntegGainShiftFW=s16IntegGainShiftQ;
      |     f16IntegGainFW=f16IntegGainQ;
      |     if (Idmax<0)
      |       iratio=abs(Idmax)/iscale;
      |       if (abs(iratio) > 1)
      |         iratio = 0;
      |       end
      |       lowlim=0.3183098861837907*acos(iratio)-0.5;
      |     else
      |       lowlim=0.0;
      |     end
      |     f16LowerLimitFW=round(lowlim*2^15);
      |     if f16LowerLimitFW>2^15-1
      |       f16LowerLimitFW=2^15-1;
      |       warning(['Parameter f16LowerLimitFW of ' gcb ' exceeds the fixed-point range.']);
      |     end
      |     if f16LowerLimitFW<-2^15
      |       f16LowerLimitFW=-2^15;
      |       warning(['Parameter f16LowerLimitFW of ' gcb ' exceeds the fixed-point range.']);
      |     end
      |     f16UpperLimitFW=0;
      |     u16NSamplesW=round(log2(1.0/abs(lambdaW)));
      |     if u16NSamplesW>15
      |       u16NSamplesW=15;
      |     end
      |     if u16NSamplesW<0
      |       u16NSamplesW=0;
      |     end
      |     u16NSamplesFW=round(log2(1.0/abs(lambdaFW)));
      |     if u16NSamplesFW>15
      |       u16NSamplesFW=15;
      |     end
      |     if u16NSamplesFW<0
      |       u16NSamplesFW=0;
      |     end
      |     rampsc=polepairs*abs(ramprpm)*0.1047197551196598/wmax;
      |     f32RampUp=round(rampsc*2^31);
      |     if f32RampUp>2^31-1
      |       f32RampUp=2^31-1;
      |       warning(['Parameter f32RampUp of ' gcb ' exceeds the fixed-point range.']);
      |     end
      |     if f32RampUp<-2^31
      |       f32RampUp=-2^31;
      |       warning(['Parameter f32RampUp of ' gcb ' exceeds the fixed-point range.']);
      |     end
      |     f32RampDown=round(rampsc*2^31);
      |     if f32RampDown>2^31-1
      |       f32RampDown=2^31-1;
      |       warning(['Parameter f32RampDown of ' gcb ' exceeds the fixed-point range.']);
      |     end
      |     if f32RampDown<-2^31
      |       f32RampDown=-2^31;
      |       warning(['Parameter f32RampDown of ' gcb ' exceeds the fixed-point range.']);
      |     end
      |     if isnan(u16NSamplesW)
      |       if ~strcmp(u16NSamplesW_bkup,'0')
      |         set_param(gcb,'u16NSamplesW','0');
      |       end
      |     else
      |       tmps=num2str(u16NSamplesW);
      |       if ~strcmp(u16NSamplesW_bkup,tmps)
      |         set_param(gcb,'u16NSamplesW',tmps);
      |       end
      |     end
      |     if isnan(u16NSamplesFW)
      |       if ~strcmp(u16NSamplesFW_bkup,'0')
      |         set_param(gcb,'u16NSamplesFW','0');
      |       end
      |     else
      |       tmps=num2str(u16NSamplesFW);
      |       if ~strcmp(u16NSamplesFW_bkup,tmps)
      |         set_param(gcb,'u16NSamplesFW',tmps);
      |       end
      |     end
      |     if isnan(f16PropGainQ)
      |       if ~strcmp(f16PropGainQ_bkup,'0')
      |         set_param(gcb,'f16PropGainQ','0');
      |       end
      |     else
      |       tmps=num2str(f16PropGainQ);
      |       if ~strcmp(f16PropGainQ_bkup,tmps)
      |         set_param(gcb,'f16PropGainQ',tmps);
      |       end
      |     end
      |     if isnan(f16IntegGainQ)
      |       if ~strcmp(f16IntegGainQ_bkup,'0')
      |         set_param(gcb,'f16IntegGainQ','0');
      |       end
      |     else
      |       tmps=num2str(f16IntegGainQ);
      |       if ~strcmp(f16IntegGainQ_bkup,tmps)
      |         set_param(gcb,'f16IntegGainQ',tmps);
      |       end
      |     end
      |     if isnan(s16PropGainShiftQ)
      |       if ~strcmp(s16PropGainShiftQ_bkup,'0')
      |         set_param(gcb,'s16PropGainShiftQ','0');
      |       end
      |     else
      |       tmps=num2str(s16PropGainShiftQ);
      |       if ~strcmp(s16PropGainShiftQ_bkup,tmps)
      |         set_param(gcb,'s16PropGainShiftQ',tmps);
      |       end
      |     end
      |     if isnan(s16IntegGainShiftQ)
      |       if ~strcmp(s16IntegGainShiftQ_bkup,'0')
      |         set_param(gcb,'s16IntegGainShiftQ','0');
      |       end
      |     else
      |       tmps=num2str(s16IntegGainShiftQ);
      |       if ~strcmp(s16IntegGainShiftQ_bkup,tmps)
      |         set_param(gcb,'s16IntegGainShiftQ',tmps);
      |       end
      |     end
      |     if isnan(f16LowerLimitQ)
      |       if ~strcmp(f16LowerLimitQ_bkup,'0')
      |         set_param(gcb,'f16LowerLimitQ','0');
      |       end
      |     else
      |       tmps=num2str(f16LowerLimitQ);
      |       if ~strcmp(f16LowerLimitQ_bkup,tmps)
      |         set_param(gcb,'f16LowerLimitQ',tmps);
      |       end
      |     end
      |     if isnan(f16UpperLimitQ)
      |       if ~strcmp(f16UpperLimitQ_bkup,'0')
      |         set_param(gcb,'f16UpperLimitQ','0');
      |       end
      |     else
      |       tmps=num2str(f16UpperLimitQ);
      |       if ~strcmp(f16UpperLimitQ_bkup,tmps)
      |         set_param(gcb,'f16UpperLimitQ',tmps);
      |       end
      |     end
      |     if isnan(f16PropGainFW)
      |       if ~strcmp(f16PropGainFW_bkup,'0')
      |         set_param(gcb,'f16PropGainFW','0');
      |       end
      |     else
      |       tmps=num2str(f16PropGainFW);
      |       if ~strcmp(f16PropGainFW_bkup,tmps)
      |         set_param(gcb,'f16PropGainFW',tmps);
      |       end
      |     end
      |     if isnan(f16IntegGainFW)
      |       if ~strcmp(f16IntegGainFW_bkup,'0')
      |         set_param(gcb,'f16IntegGainFW','0');
      |       end
      |     else
      |       tmps=num2str(f16IntegGainFW);
      |       if ~strcmp(f16IntegGainFW_bkup,tmps)
      |         set_param(gcb,'f16IntegGainFW',tmps);
      |       end
      |     end
      |     if isnan(s16PropGainShiftFW)
      |       if ~strcmp(s16PropGainShiftFW_bkup,'0')
      |         set_param(gcb,'s16PropGainShiftFW','0');
      |       end
      |     else
      |       tmps=num2str(s16PropGainShiftFW);
      |       if ~strcmp(s16PropGainShiftFW_bkup,tmps)
      |         set_param(gcb,'s16PropGainShiftFW',tmps);
      |       end
      |     end
      |     if isnan(s16IntegGainShiftFW)
      |       if ~strcmp(s16IntegGainShiftFW_bkup,'0')
      |         set_param(gcb,'s16IntegGainShiftFW','0');
      |       end
      |     else
      |       tmps=num2str(s16IntegGainShiftFW);
      |       if ~strcmp(s16IntegGainShiftFW_bkup,tmps)
      |         set_param(gcb,'s16IntegGainShiftFW',tmps);
      |       end
      |     end
      |     if isnan(f16LowerLimitFW)
      |       if ~strcmp(f16LowerLimitFW_bkup,'0')
      |         set_param(gcb,'f16LowerLimitFW','0');
      |       end
      |     else
      |       tmps=num2str(f16LowerLimitFW);
      |       if ~strcmp(f16LowerLimitFW_bkup,tmps)
      |         set_param(gcb,'f16LowerLimitFW',tmps);
      |       end
      |     end
      |     if isnan(f16UpperLimitFW)
      |       if ~strcmp(f16UpperLimitFW_bkup,'0')
      |         set_param(gcb,'f16UpperLimitFW','0');
      |       end
      |     else
      |       tmps=num2str(f16UpperLimitFW);
      |       if ~strcmp(f16UpperLimitFW_bkup,tmps)
      |         set_param(gcb,'f16UpperLimitFW',tmps);
      |       end
      |     end
      |     if isnan(f32RampUp)
      |       if ~strcmp(f32RampUp_bkup,'0')
      |         set_param(gcb,'f32RampUp','0');
      |       end
      |     else
      |       tmps=num2str(f32RampUp);
      |       if ~strcmp(f32RampUp_bkup,tmps)
      |         set_param(gcb,'f32RampUp',tmps);
      |       end
      |     end
      |     if isnan(f32RampDown)
      |       if ~strcmp(f32RampDown_bkup,'0')
      |         set_param(gcb,'f32RampDown','0');
      |       end
      |     else
      |       tmps=num2str(f32RampDown);
      |       if ~strcmp(f32RampDown_bkup,tmps)
      |         set_param(gcb,'f32RampDown',tmps);
      |       end
      |     end
      |   end
      | end
      mask Callback wf0:
      | autoCalcEn=get_param(gcb,'autoCalcEn');
      | if strcmp(autoCalcEn,'on')
      |   SampleTime=Simulink.data.evalinGlobal(bdroot,get_param(gcb,'SampleTime'));
      |   if (SampleTime==-1)
      |     SampleTime=str2double(get_param(gcb,'SampleTime_1'));
      |   end
      |   u16NSamplesW_bkup=get_param(gcb,'u16NSamplesW');
      |   u16NSamplesFW_bkup=get_param(gcb,'u16NSamplesFW');
      |   f16PropGainQ_bkup=get_param(gcb,'f16PropGainQ');
      |   f16IntegGainQ_bkup=get_param(gcb,'f16IntegGainQ');
      |   s16PropGainShiftQ_bkup=get_param(gcb,'s16PropGainShiftQ');
      |   s16IntegGainShiftQ_bkup=get_param(gcb,'s16IntegGainShiftQ');
      |   f16LowerLimitQ_bkup=get_param(gcb,'f16LowerLimitQ');
      |   f16UpperLimitQ_bkup=get_param(gcb,'f16UpperLimitQ');
      |   f16PropGainFW_bkup=get_param(gcb,'f16PropGainFW');
      |   f16IntegGainFW_bkup=get_param(gcb,'f16IntegGainFW');
      |   s16PropGainShiftFW_bkup=get_param(gcb,'s16PropGainShiftFW');
      |   s16IntegGainShiftFW_bkup=get_param(gcb,'s16IntegGainShiftFW');
      |   f16LowerLimitFW_bkup=get_param(gcb,'f16LowerLimitFW');
      |   f16UpperLimitFW_bkup=get_param(gcb,'f16UpperLimitFW');
      |   f32RampUp_bkup=get_param(gcb,'f32RampUp');
      |   f32RampDown_bkup=get_param(gcb,'f32RampDown');
      |   wf0=Simulink.data.evalinGlobal(bdroot,get_param(gcb,'wf0'));
      |   wksi=Simulink.data.evalinGlobal(bdroot,get_param(gcb,'wksi'));
      |   J=Simulink.data.evalinGlobal(bdroot,get_param(gcb,'J'));
      |   Kt=Simulink.data.evalinGlobal(bdroot,get_param(gcb,'Kt'));
      |   lambdaW=Simulink.data.evalinGlobal(bdroot,get_param(gcb,'lambdaW'));
      |   lambdaFW=Simulink.data.evalinGlobal(bdroot,get_param(gcb,'lambdaFW'));
      |   Idmax=Simulink.data.evalinGlobal(bdroot,get_param(gcb,'Idmax'));
      |   ramprpm=Simulink.data.evalinGlobal(bdroot,get_param(gcb,'ramprpm'));
      |   mechspeed=Simulink.data.evalinGlobal(bdroot,get_param(gcb,'mechspeed'));
      |   polepairs=Simulink.data.evalinGlobal(bdroot,get_param(gcb,'polepairs'));
      |   uscale=Simulink.data.evalinGlobal(bdroot,get_param(gcb,'uscale'));
      |   iscale=Simulink.data.evalinGlobal(bdroot,get_param(gcb,'iscale'));
      |   if (wf0<=0)
      |     warning('Natural frequency f0 must be positive.');
      |   end
      |   if (wksi<=0)
      |     warning('Current loop attenuation must be positive.');
      |   end
      |   if (wksi>1)
      |     warning('Current loop attenuation must not exceed 1.');
      |   end
      |   if (J<=0)
      |     warning('Moment of inertia J must be positive.');
      |   end
      |   if (Kt<=0)
      |     warning('Torque constant Kt must be positive.');
      |   end
      |   if (lambdaW<0)
      |     warning('MA filter smoothing factor must be in the range 0..1.');
      |   end
      |   if (lambdaW>1)
      |     warning('MA filter smoothing factor must be in the range 0..1.');
      |   end
      |   if (lambdaFW<0)
      |     warning('MA filter smoothing factor must be in the range 0..1.');
      |   end
      |   if (lambdaFW>1)
      |     warning('MA filter smoothing factor must be in the range 0..1.');
      |   end
      |   if (mechspeed<=0)
      |     warning('Max. speed must be positive.');
      |   end
      |   if (polepairs<1)
      |     warning('Number of pole pairs must be a natural number (1, 2, 3, ...).');
      |   end
      |   if (round(polepairs)~=polepairs)
      |     warning('Number of pole pairs must be a natural number (1, 2, 3, ...).');
      |   end
      |   if (uscale<=0)
      |     warning('U_max must be positive.');
      |   end
      |   if (iscale<=0)
      |     warning('I_max must be positive.');
      |   end
      |   w0=6.283185307179586*wf0;
      |   pgain=2.0*wksi*w0*J/Kt;
      |   igain=w0*w0*J/Kt;
      |   wmax=polepairs*mechspeed*0.1047197551196598;
      |   kpf=pgain*wmax/iscale;
      |   s16PropGainShiftQ=ceil(log2(abs(kpf)));
      |   if s16PropGainShiftQ<-15
      |     s16PropGainShiftQ=-15;
      |   end
      |   if s16PropGainShiftQ>15
      |     s16PropGainShiftQ=15;
      |     warning(['Parameter s16PropGainShiftQ of ' gcb ' exceeds the fixed-point range.']);
      |   end
      |   f16PropGainQ=round(kpf*2^(-s16PropGainShiftQ)*2^15);
      |   if f16PropGainQ>2^15-1
      |     f16PropGainQ=2^15-1;
      |     warning(['Parameter f16PropGainQ of ' gcb ' exceeds the fixed-point range.']);
      |   end
      |   if f16PropGainQ<-2^15
      |     f16PropGainQ=-2^15;
      |     warning(['Parameter f16PropGainQ of ' gcb ' exceeds the fixed-point range.']);
      |   end
      |   kif=igain*SampleTime*0.5*wmax/iscale;
      |   s16IntegGainShiftQ=ceil(log2(abs(kif)));
      |   if s16IntegGainShiftQ<-15
      |     s16IntegGainShiftQ=-15;
      |   end
      |   if s16IntegGainShiftQ>15
      |     s16IntegGainShiftQ=15;
      |     warning(['Parameter s16IntegGainShiftQ of ' gcb ' exceeds the fixed-point range.']);
      |   end
      |   f16IntegGainQ=round(kif*2^(-s16IntegGainShiftQ)*2^15);
      |   if f16IntegGainQ>2^15-1
      |     f16IntegGainQ=2^15-1;
      |     warning(['Parameter f16IntegGainQ of ' gcb ' exceeds the fixed-point range.']);
      |   end
      |   if f16IntegGainQ<-2^15
      |     f16IntegGainQ=-2^15;
      |     warning(['Parameter f16IntegGainQ of ' gcb ' exceeds the fixed-point range.']);
      |   end
      |   f16LowerLimitQ=-32768;
      |   f16UpperLimitQ=32767;
      |   fwkpf=0.9*pgain*wmax/iscale;
      |   s16PropGainShiftFW=ceil(log2(abs(fwkpf)));
      |   if s16PropGainShiftFW<-15
      |     s16PropGainShiftFW=-15;
      |   end
      |   if s16PropGainShiftFW>15
      |     s16PropGainShiftFW=15;
      |     warning(['Parameter s16PropGainShiftFW of ' gcb ' exceeds the fixed-point range.']);
      |   end
      |   f16PropGainFW=round(fwkpf*2^(-s16PropGainShiftFW)*2^15);
      |   if f16PropGainFW>2^15-1
      |     f16PropGainFW=2^15-1;
      |     warning(['Parameter f16PropGainFW of ' gcb ' exceeds the fixed-point range.']);
      |   end
      |   if f16PropGainFW<-2^15
      |     f16PropGainFW=-2^15;
      |     warning(['Parameter f16PropGainFW of ' gcb ' exceeds the fixed-point range.']);
      |   end
      |   s16IntegGainShiftFW=s16IntegGainShiftQ;
      |   f16IntegGainFW=f16IntegGainQ;
      |   if (Idmax<0)
      |     iratio=abs(Idmax)/iscale;
      |     if (abs(iratio) > 1)
      |       iratio = 0;
      |     end
      |     lowlim=0.3183098861837907*acos(iratio)-0.5;
      |   else
      |     lowlim=0.0;
      |   end
      |   f16LowerLimitFW=round(lowlim*2^15);
      |   if f16LowerLimitFW>2^15-1
      |     f16LowerLimitFW=2^15-1;
      |     warning(['Parameter f16LowerLimitFW of ' gcb ' exceeds the fixed-point range.']);
      |   end
      |   if f16LowerLimitFW<-2^15
      |     f16LowerLimitFW=-2^15;
      |     warning(['Parameter f16LowerLimitFW of ' gcb ' exceeds the fixed-point range.']);
      |   end
      |   f16UpperLimitFW=0;
      |   u16NSamplesW=round(log2(1.0/abs(lambdaW)));
      |   if u16NSamplesW>15
      |     u16NSamplesW=15;
      |   end
      |   if u16NSamplesW<0
      |     u16NSamplesW=0;
      |   end
      |   u16NSamplesFW=round(log2(1.0/abs(lambdaFW)));
      |   if u16NSamplesFW>15
      |     u16NSamplesFW=15;
      |   end
      |   if u16NSamplesFW<0
      |     u16NSamplesFW=0;
      |   end
      |   rampsc=polepairs*abs(ramprpm)*0.1047197551196598/wmax;
      |   f32RampUp=round(rampsc*2^31);
      |   if f32RampUp>2^31-1
      |     f32RampUp=2^31-1;
      |     warning(['Parameter f32RampUp of ' gcb ' exceeds the fixed-point range.']);
      |   end
      |   if f32RampUp<-2^31
      |     f32RampUp=-2^31;
      |     warning(['Parameter f32RampUp of ' gcb ' exceeds the fixed-point range.']);
      |   end
      |   f32RampDown=round(rampsc*2^31);
      |   if f32RampDown>2^31-1
      |     f32RampDown=2^31-1;
      |     warning(['Parameter f32RampDown of ' gcb ' exceeds the fixed-point range.']);
      |   end
      |   if f32RampDown<-2^31
      |     f32RampDown=-2^31;
      |     warning(['Parameter f32RampDown of ' gcb ' exceeds the fixed-point range.']);
      |   end
      |   if isnan(u16NSamplesW)
      |     if ~strcmp(u16NSamplesW_bkup,'0')
      |       set_param(gcb,'u16NSamplesW','0');
      |     end
      |   else
      |     tmps=num2str(u16NSamplesW);
      |     if ~strcmp(u16NSamplesW_bkup,tmps)
      |       set_param(gcb,'u16NSamplesW',tmps);
      |     end
      |   end
      |   if isnan(u16NSamplesFW)
      |     if ~strcmp(u16NSamplesFW_bkup,'0')
      |       set_param(gcb,'u16NSamplesFW','0');
      |     end
      |   else
      |     tmps=num2str(u16NSamplesFW);
      |     if ~strcmp(u16NSamplesFW_bkup,tmps)
      |       set_param(gcb,'u16NSamplesFW',tmps);
      |     end
      |   end
      |   if isnan(f16PropGainQ)
      |     if ~strcmp(f16PropGainQ_bkup,'0')
      |       set_param(gcb,'f16PropGainQ','0');
      |     end
      |   else
      |     tmps=num2str(f16PropGainQ);
      |     if ~strcmp(f16PropGainQ_bkup,tmps)
      |       set_param(gcb,'f16PropGainQ',tmps);
      |     end
      |   end
      |   if isnan(f16IntegGainQ)
      |     if ~strcmp(f16IntegGainQ_bkup,'0')
      |       set_param(gcb,'f16IntegGainQ','0');
      |     end
      |   else
      |     tmps=num2str(f16IntegGainQ);
      |     if ~strcmp(f16IntegGainQ_bkup,tmps)
      |       set_param(gcb,'f16IntegGainQ',tmps);
      |     end
      |   end
      |   if isnan(s16PropGainShiftQ)
      |     if ~strcmp(s16PropGainShiftQ_bkup,'0')
      |       set_param(gcb,'s16PropGainShiftQ','0');
      |     end
      |   else
      |     tmps=num2str(s16PropGainShiftQ);
      |     if ~strcmp(s16PropGainShiftQ_bkup,tmps)
      |       set_param(gcb,'s16PropGainShiftQ',tmps);
      |     end
      |   end
      |   if isnan(s16IntegGainShiftQ)
      |     if ~strcmp(s16IntegGainShiftQ_bkup,'0')
      |       set_param(gcb,'s16IntegGainShiftQ','0');
      |     end
      |   else
      |     tmps=num2str(s16IntegGainShiftQ);
      |     if ~strcmp(s16IntegGainShiftQ_bkup,tmps)
      |       set_param(gcb,'s16IntegGainShiftQ',tmps);
      |     end
      |   end
      |   if isnan(f16LowerLimitQ)
      |     if ~strcmp(f16LowerLimitQ_bkup,'0')
      |       set_param(gcb,'f16LowerLimitQ','0');
      |     end
      |   else
      |     tmps=num2str(f16LowerLimitQ);
      |     if ~strcmp(f16LowerLimitQ_bkup,tmps)
      |       set_param(gcb,'f16LowerLimitQ',tmps);
      |     end
      |   end
      |   if isnan(f16UpperLimitQ)
      |     if ~strcmp(f16UpperLimitQ_bkup,'0')
      |       set_param(gcb,'f16UpperLimitQ','0');
      |     end
      |   else
      |     tmps=num2str(f16UpperLimitQ);
      |     if ~strcmp(f16UpperLimitQ_bkup,tmps)
      |       set_param(gcb,'f16UpperLimitQ',tmps);
      |     end
      |   end
      |   if isnan(f16PropGainFW)
      |     if ~strcmp(f16PropGainFW_bkup,'0')
      |       set_param(gcb,'f16PropGainFW','0');
      |     end
      |   else
      |     tmps=num2str(f16PropGainFW);
      |     if ~strcmp(f16PropGainFW_bkup,tmps)
      |       set_param(gcb,'f16PropGainFW',tmps);
      |     end
      |   end
      |   if isnan(f16IntegGainFW)
      |     if ~strcmp(f16IntegGainFW_bkup,'0')
      |       set_param(gcb,'f16IntegGainFW','0');
      |     end
      |   else
      |     tmps=num2str(f16IntegGainFW);
      |     if ~strcmp(f16IntegGainFW_bkup,tmps)
      |       set_param(gcb,'f16IntegGainFW',tmps);
      |     end
      |   end
      |   if isnan(s16PropGainShiftFW)
      |     if ~strcmp(s16PropGainShiftFW_bkup,'0')
      |       set_param(gcb,'s16PropGainShiftFW','0');
      |     end
      |   else
      |     tmps=num2str(s16PropGainShiftFW);
      |     if ~strcmp(s16PropGainShiftFW_bkup,tmps)
      |       set_param(gcb,'s16PropGainShiftFW',tmps);
      |     end
      |   end
      |   if isnan(s16IntegGainShiftFW)
      |     if ~strcmp(s16IntegGainShiftFW_bkup,'0')
      |       set_param(gcb,'s16IntegGainShiftFW','0');
      |     end
      |   else
      |     tmps=num2str(s16IntegGainShiftFW);
      |     if ~strcmp(s16IntegGainShiftFW_bkup,tmps)
      |       set_param(gcb,'s16IntegGainShiftFW',tmps);
      |     end
      |   end
      |   if isnan(f16LowerLimitFW)
      |     if ~strcmp(f16LowerLimitFW_bkup,'0')
      |       set_param(gcb,'f16LowerLimitFW','0');
      |     end
      |   else
      |     tmps=num2str(f16LowerLimitFW);
      |     if ~strcmp(f16LowerLimitFW_bkup,tmps)
      |       set_param(gcb,'f16LowerLimitFW',tmps);
      |     end
      |   end
      |   if isnan(f16UpperLimitFW)
      |     if ~strcmp(f16UpperLimitFW_bkup,'0')
      |       set_param(gcb,'f16UpperLimitFW','0');
      |     end
      |   else
      |     tmps=num2str(f16UpperLimitFW);
      |     if ~strcmp(f16UpperLimitFW_bkup,tmps)
      |       set_param(gcb,'f16UpperLimitFW',tmps);
      |     end
      |   end
      |   if isnan(f32RampUp)
      |     if ~strcmp(f32RampUp_bkup,'0')
      |       set_param(gcb,'f32RampUp','0');
      |     end
      |   else
      |     tmps=num2str(f32RampUp);
      |     if ~strcmp(f32RampUp_bkup,tmps)
      |       set_param(gcb,'f32RampUp',tmps);
      |     end
      |   end
      |   if isnan(f32RampDown)
      |     if ~strcmp(f32RampDown_bkup,'0')
      |       set_param(gcb,'f32RampDown','0');
      |     end
      |   else
      |     tmps=num2str(f32RampDown);
      |     if ~strcmp(f32RampDown_bkup,tmps)
      |       set_param(gcb,'f32RampDown',tmps);
      |     end
      |   end
      | end
      mask Callback wksi:
      | autoCalcEn=get_param(gcb,'autoCalcEn');
      | if strcmp(autoCalcEn,'on')
      |   SampleTime=Simulink.data.evalinGlobal(bdroot,get_param(gcb,'SampleTime'));
      |   if (SampleTime==-1)
      |     SampleTime=str2double(get_param(gcb,'SampleTime_1'));
      |   end
      |   u16NSamplesW_bkup=get_param(gcb,'u16NSamplesW');
      |   u16NSamplesFW_bkup=get_param(gcb,'u16NSamplesFW');
      |   f16PropGainQ_bkup=get_param(gcb,'f16PropGainQ');
      |   f16IntegGainQ_bkup=get_param(gcb,'f16IntegGainQ');
      |   s16PropGainShiftQ_bkup=get_param(gcb,'s16PropGainShiftQ');
      |   s16IntegGainShiftQ_bkup=get_param(gcb,'s16IntegGainShiftQ');
      |   f16LowerLimitQ_bkup=get_param(gcb,'f16LowerLimitQ');
      |   f16UpperLimitQ_bkup=get_param(gcb,'f16UpperLimitQ');
      |   f16PropGainFW_bkup=get_param(gcb,'f16PropGainFW');
      |   f16IntegGainFW_bkup=get_param(gcb,'f16IntegGainFW');
      |   s16PropGainShiftFW_bkup=get_param(gcb,'s16PropGainShiftFW');
      |   s16IntegGainShiftFW_bkup=get_param(gcb,'s16IntegGainShiftFW');
      |   f16LowerLimitFW_bkup=get_param(gcb,'f16LowerLimitFW');
      |   f16UpperLimitFW_bkup=get_param(gcb,'f16UpperLimitFW');
      |   f32RampUp_bkup=get_param(gcb,'f32RampUp');
      |   f32RampDown_bkup=get_param(gcb,'f32RampDown');
      |   wf0=Simulink.data.evalinGlobal(bdroot,get_param(gcb,'wf0'));
      |   wksi=Simulink.data.evalinGlobal(bdroot,get_param(gcb,'wksi'));
      |   J=Simulink.data.evalinGlobal(bdroot,get_param(gcb,'J'));
      |   Kt=Simulink.data.evalinGlobal(bdroot,get_param(gcb,'Kt'));
      |   lambdaW=Simulink.data.evalinGlobal(bdroot,get_param(gcb,'lambdaW'));
      |   lambdaFW=Simulink.data.evalinGlobal(bdroot,get_param(gcb,'lambdaFW'));
      |   Idmax=Simulink.data.evalinGlobal(bdroot,get_param(gcb,'Idmax'));
      |   ramprpm=Simulink.data.evalinGlobal(bdroot,get_param(gcb,'ramprpm'));
      |   mechspeed=Simulink.data.evalinGlobal(bdroot,get_param(gcb,'mechspeed'));
      |   polepairs=Simulink.data.evalinGlobal(bdroot,get_param(gcb,'polepairs'));
      |   uscale=Simulink.data.evalinGlobal(bdroot,get_param(gcb,'uscale'));
      |   iscale=Simulink.data.evalinGlobal(bdroot,get_param(gcb,'iscale'));
      |   if (wf0<=0)
      |     warning('Natural frequency f0 must be positive.');
      |   end
      |   if (wksi<=0)
      |     warning('Current loop attenuation must be positive.');
      |   end
      |   if (wksi>1)
      |     warning('Current loop attenuation must not exceed 1.');
      |   end
      |   if (J<=0)
      |     warning('Moment of inertia J must be positive.');
      |   end
      |   if (Kt<=0)
      |     warning('Torque constant Kt must be positive.');
      |   end
      |   if (lambdaW<0)
      |     warning('MA filter smoothing factor must be in the range 0..1.');
      |   end
      |   if (lambdaW>1)
      |     warning('MA filter smoothing factor must be in the range 0..1.');
      |   end
      |   if (lambdaFW<0)
      |     warning('MA filter smoothing factor must be in the range 0..1.');
      |   end
      |   if (lambdaFW>1)
      |     warning('MA filter smoothing factor must be in the range 0..1.');
      |   end
      |   if (mechspeed<=0)
      |     warning('Max. speed must be positive.');
      |   end
      |   if (polepairs<1)
      |     warning('Number of pole pairs must be a natural number (1, 2, 3, ...).');
      |   end
      |   if (round(polepairs)~=polepairs)
      |     warning('Number of pole pairs must be a natural number (1, 2, 3, ...).');
      |   end
      |   if (uscale<=0)
      |     warning('U_max must be positive.');
      |   end
      |   if (iscale<=0)
      |     warning('I_max must be positive.');
      |   end
      |   w0=6.283185307179586*wf0;
      |   pgain=2.0*wksi*w0*J/Kt;
      |   igain=w0*w0*J/Kt;
      |   wmax=polepairs*mechspeed*0.1047197551196598;
      |   kpf=pgain*wmax/iscale;
      |   s16PropGainShiftQ=ceil(log2(abs(kpf)));
      |   if s16PropGainShiftQ<-15
      |     s16PropGainShiftQ=-15;
      |   end
      |   if s16PropGainShiftQ>15
      |     s16PropGainShiftQ=15;
      |     warning(['Parameter s16PropGainShiftQ of ' gcb ' exceeds the fixed-point range.']);
      |   end
      |   f16PropGainQ=round(kpf*2^(-s16PropGainShiftQ)*2^15);
      |   if f16PropGainQ>2^15-1
      |     f16PropGainQ=2^15-1;
      |     warning(['Parameter f16PropGainQ of ' gcb ' exceeds the fixed-point range.']);
      |   end
      |   if f16PropGainQ<-2^15
      |     f16PropGainQ=-2^15;
      |     warning(['Parameter f16PropGainQ of ' gcb ' exceeds the fixed-point range.']);
      |   end
